simulink library "AEMS_Standard_Library"  (R2016b)
settings: Solver=ode45  StartTime=0.0  StopTime=10.0  RelTol=1e-3
undefined symbols (not defined in the file or in its folder): BkPY, carto, Cbx_extegr, Cbx_lpegrsys, Cbx_portegr, Cnx_bnk_nr_conf, Cnx_cyl_nr_conf, ConfigManagement, configuration_management, Cxx_dcm_io_tmr_end_xxxx, Cxx_dcm_rt_tmr_end, Cxx_DID_xxxx_IO_max, Cxx_DID_xxxx_IO_min, Cxx_egrhsofs, Cxx_vmaniegi, DEM_DEBOUNCE_FREEZE, DEM_DTR_CTL_INVISIBLE, DEM_DTR_CTL_NORMAL, Dem_DtrId2_XXX, Dem_DtrId3_XXX, Dem_DtrId4_XXX, Dem_DtrId5_XXX, Dem_DtrId6_XXX, Dem_DtrId7_XXX, Dem_DtrId8_XXX, Dem_DtrId9_XXX, Dem_DtrId_XXX, Dem_EnableConditionId2_XXX, Dem_EnableConditionId3_XXX, Dem_EnableConditionId4_XXX, Dem_EnableConditionId5_XXX, Dem_EnableConditionId6_XXX, Dem_EnableConditionId7_XXX, Dem_EnableConditionId8_XXX, Dem_EnableConditionId_XXX, Dem_EventId, Dem_EventId2_XXX, Dem_EventId3_XXX, Dem_EventId4_XXX, Dem_EventId5_XXX, Dem_EventId6_XXX, Dem_EventId7_XXX, Dem_EventId8_XXX, Dem_EventId9_XXX, Dem_EventId_Device_Faulttype, Dem_EventId_XXX, DEM_IUMPR_GENERAL_DENOMINATOR, DEM_OPCYC_IGNITION, Dem_RatioId2_XXX, Dem_RatioId3_XXX, Dem_RatioId4_XXX, Dem_RatioId5_XXX, Dem_RatioId6_XXX, Dem_RatioId7_XXX, Dem_RatioId8_XXX, Dem_RatioId_XXX, Dem_StorageConditionId2_XXX, Dem_StorageConditionId3_XXX, Dem_StorageConditionId4_XXX, Dem_StorageConditionId5_XXX ... (+65)
libraries: AEMS_Standard_Library x477, simulink x2
(part 6 of 39)

== system AEMS_Standard_Library/DEM ==
  note: AUTOSAR IN
  note: AUTOSAR OUT
  note: FIM
  note: NISSAN USES
  AEMS_DEM_COUNTER_BASED_DEBOUNCE : Subsystem  Tag=[LIB]  Description=This subsystem is interface for self diagnosis standard calculated from similar condition and NG judgment.  mask(AEMS_DEM_COUNTER_BASED_DEBOUNCE){eventid=Dem_EventId_Device_Faulttype, Specificchoix=off, Dim_num=1, DemDebounceBehavior1=DEM_DEBOUNCE_FREEZE (0), DemDebounceBehavior2=DEM_DEBOUNCE_FREEZE (0), DemDebounceBehavior3=DEM_DEBOUNCE_FREEZE (0), DemDebounceBehavior4=DEM_DEBOUNCE_FREEZE (0), DemDebounceBehavior5=DEM_DEBOUNCE_FREEZE (0), DemDebounceBehavior6=DEM_DEBOUNCE_FREEZE (0), DemDebounceBehavior7=DEM_DEBOUNCE_FREEZE (0), DemDebounceBehavior8=DEM_DEBOUNCE_FREEZE (0), DemCounterFailedThreshold=Cnx_dem_fail_thd_Device_Faulttype, DemCounterIncrementStepSize=Cnx_dem_pfail_inc_step_Device_Faulttype, DemCounterJumpUp=Cbx_dem_jmp_up_act_Device_Faulttype, DemCounterJumpUpValue=Cnx_dem_jmp_up_pfail_Device_Faulttype, DemCounterPassedThreshold=Cnx_dem_pass_thd_Device_Faulttype, DemCounterDecrementStepSize=Cnx_dem_ppass_dec_step_Device_Faulttype, DemCounterJumpDown=Cbx_dem_jmp_dwn_act_Device_Faulttype, DemCounterJumpDownValue=Cnx_dem_jmp_dwn_ppass_Device_Faulttype, DemCounterBypassFailure=Cbx_dem_byp_fail_Device_Faulttype, ToDataStoreMemory=off}
      mask prompts: eventid "Identifier of a diagnostic event (EventId)"; Specificchoix "Specific case used only for Nissan cases"; Dim_num "Dimension :"; DemDebounceBehavior1 "Dem Debounce Behavior 1"; DemDebounceBehavior2 "Dem Debounce Behavior 2"; DemDebounceBehavior3 "Dem Debounce Behavior 3"; DemDebounceBehavior4 "Dem Debounce Behavior 4"; DemDebounceBehavior5 "Dem Debounce Behavior 5"; DemDebounceBehavior6 "Dem Debounce Behavior 6"; DemDebounceBehavior7 "Dem Debounce Behavior 7"; DemDebounceBehavior8 "Dem Debounce Behavior 8"; DemCounterFailedThreshold "Dem Debounce Counter Failed Threshold"; DemCounterIncrementStepSize "Dem Debounce Counter Increment Step Size"; DemCounterJumpUp "Dem Debounce Counter Jump Up"; DemCounterJumpUpValue "Dem Debounce Counter Jump Up Value"; DemCounterPassedThreshold "Dem Debounce Counter Passed Threshold"; DemCounterDecrementStepSize "Dem Debounce Counter Decrement Step Size"; DemCounterJumpDown "Dem Debounce Counter Jump Down"; DemCounterJumpDownValue "Dem Debounce Counter Jump Down Value"; DemCounterBypassFailure "Dem Debounce Counter Bypass Failure"; ToDataStoreMemory "Write Output To Data Store Memory"
      mask help:
      | It  transmit the status Failed or Passed to the DEM. Accordingly, some bits of the UDS DTC status byte changes synchronously or asynchronously according to the configuration. Debounce is based on counter.
      |
      | -INPUTS-
      | conditionfulfilled: specifies whether the storage condition assigned to the StorageConditionId is fulfilled
      | prefailed: Monitor reports nonqualified test result pre-failed
      | prepassed: Monitor reports nonqualified test result pre-passed
      | ClearDataRequest:Clears the Data Request value
      | reseteventdebounce: Freeze or reset the internal debounce counter/timer.
      |
      | -OUTPUTS-
      | debouncevalue: Value of the debounce counter
      | failed: Diagnostic monitor reports an event Failed
      | passed: Diagnostic monitor reports an event passed
      |
      | -PARAMETERS-
      | Device: Device type
      | FaultType: Fault Type
      | EventId: Internal identifier of a diagnostic event. 0 is not a valid value.
      | Dem Debounce Behavior: The event debounce counter will be frozen or reset (0 for FREEZE and 1 for RESET)
      | Dem Debounce Counter Failed Threshold: Defines the value of the internal debounce counter, which indicates the failed status.
      | Dem Debounce Counter Increment Step Size: Defines the incrementation  step size for counter (PREFAILED)
      | Dem Debounce Counter Jump Up: Activation of Jump-Up. True: activated. False: deactivated
      | Dem Debounce Counter Jump Up Value: Initialization value for the counter when PREFAILED
      | Dem Debounce Counter Passed Threshold: Defines the value of the internal debounce counter, which indicates the passed status.
      | Dem Debounce Counter Decrement Step Size: Defines the decrementation step for of counter (PREPASSED).
      | Dem Debounce Counter Jump Down: Activation of Jump-Down. True: Jump-Down activated
      | Dem Debounce Counter Jump Down Value: Initialization value for the counter when PREPASSED
      mask init:
      | lib_path = gcb;
      | child_lib = find_system(lib_path,'LookUnderMasks','all','FollowLinks','on','Name','AEMS_DEM_COUNTER_BASED_DEBOUNCE_D');
      | Attribute_Format_String_Part1 = '%<MaskType>\n EventId : = %<eventid> \n Specific case used only for Nissan cases := %<Specificchoix> ';
      | Attribute_Format_String_Part2 = '';
      | if strcmpi(Specificchoix,'off')
      |     Dim_num = '1';
      | else
      |     Attribute_Format_String_Part2 = '\n Dimension := %<Dim_num> ';
      | end
      | dim_block = ['AEMS_DEM_COUNTER_BASED_DEBOUNCE_' Dim_num 'D'];
      | 
      | rep_block = ['AEMS_Standard_Library/SUB/',dim_block];
      | if ismember(get_param(child_lib,'MaskType'),{dim_block})
      | else
      |     replace_block(lib_path,'FollowLinks','on','Name','AEMS_DEM_COUNTER_BASED_DEBOUNCE_D',rep_block,'noprompt');
      | end
      | 
      | Attribute_Format_String_Part3='';
      | for i=1:str2num(Dim_num)
      |     Attribute_Format_String_Part3=[Attribute_Format_String_Part3,'\n Dem Debounce Behavior ',num2str(i),' := %<DemDebounceBehavior',num2str(i),'>'];
      |     set_param([child_lib{:}],['DemDebounceBehavior',num2str(i)],get_param(lib_path,['DemDebounceBehavior',num2str(i)]));
      | end
      | 
      | if 1
      |     DemCounterFailedThreshold_tmp = get_param(lib_path,'DemCounterFailedThreshold');
      |     DemCounterIncrementStepSize_tmp = get_param(lib_path,'DemCounterIncrementStepSize');
      |     DemCounterJumpUp_tmp = get_param(lib_path,'DemCounterJumpUp');
      |     DemCounterJumpUpValue_tmp = get_param(lib_path,'DemCounterJumpUpValue');
      |     DemCounterPassedThreshold_tmp = get_param(lib_path,'DemCounterPassedThreshold');
      |     DemCounterDecrementStepSize_tmp = get_param(lib_path,'DemCounterDecrementStepSize');
      |     DemCounterJumpDown_tmp = get_param(lib_path,'DemCounterJumpDown');
      |     DemCounterJumpDownValue_tmp = get_param(lib_path,'DemCounterJumpDownValue');
      |     DemCounterBypassFailure_tmp = get_param(lib_path,'DemCounterBypassFailure');
      |     
      |     set_param([child_lib{:}],'eventid',eventid);
      |     set_param([child_lib{:}],'DemCounterFailedThreshold',DemCounterFailedThreshold_tmp);
      |     set_param([child_lib{:}],'DemCounterIncrementStepSize',DemCounterIncrementStepSize_tmp);
      |     set_param([child_lib{:}],'DemCounterJumpUp',DemCounterJumpUp_tmp);
      |     set_param([child_lib{:}],'DemCounterJumpUpValue',DemCounterJumpUpValue_tmp);
      |     set_param([child_lib{:}],'DemCounterPassedThreshold',DemCounterPassedThreshold_tmp);
      |     set_param([child_lib{:}],'DemCounterDecrementStepSize',DemCounterDecrementStepSize_tmp);
      |     set_param([child_lib{:}],'DemCounterJumpDown',DemCounterJumpDown_tmp);
      |     set_param([child_lib{:}],'DemCounterJumpDownValue',DemCounterJumpDownValue_tmp);
      |     set_param([child_lib{:}],'DemCounterBypassFailure',DemCounterBypassFailure_tmp);
      | else
      |     %do nothing
      | end
      | 
      | %If To DataStoreMemory is enabled...
      | 
      | if strcmpi(ToDataStoreMemory,'on')&& isempty(find_system(lib_path,'LookUnderMasks','all','FollowLinks','on','Name','AEMS_SRFLIPFLOP'))
      |     add_block('AEMS_Standard_Library/FLAG/AEMS_SRFLIPFLOP',[lib_path,'/AEMS_SRFLIPFLOP'],'Position',[995 224 1080 346]);
      |     add_block('simulink/Signal Attributes/Data Type Conversion',[lib_path,'/Data Type Conversion'],'Position',[1145 273 1200 297],'ShowName','off');
      |     add_block('simulink/Signal Routing/Data Store Write',[lib_path,'/Data Store Write'],'Position',[1250 272 1475 298],'ShowName','off');
      |     add_line(lib_path,'AEMS_DEM_COUNTER_BASED_DEBOUNCE_D/2','AEMS_SRFLIPFLOP/1','AutoRouting','on');
      |     add_line(lib_path,'AEMS_DEM_COUNTER_BASED_DEBOUNCE_D/3','AEMS_SRFLIPFLOP/2','AutoRouting','on');
      |     add_line(lib_path,'AEMS_SRFLIPFLOP/1','Data Type Conversion/1');
      |     add_line(lib_path,'Data Type Conversion/1','Data Store Write/1');
      | elseif strcmpi(ToDataStoreMemory,'off') && ~isempty(find_system(lib_path,'LookUnderMasks','all','FollowLinks','on','Name','AEMS_SRFLIPFLOP'))
      |     delete_block([lib_path,'/Data Type Conversion']);
      |     delete_block([lib_path,'/Data Store Write']);
      |     delete_block([lib_path,'/AEMS_SRFLIPFLOP']);
      |     delete_line(find_system(lib_path,'FollowLinks','on','FindAll','on','LookUnderMasks','on','Type','line','Connected','off'));
      | end
      | if strcmpi(ToDataStoreMemory,'on')
      |     %Get Task Rate of this block.(As per AEMS arch, all the blks shall be
      |     %kept under the runnable. The Runnable name will ncontain the sample
      |     %time suffix. From where we can get it.
      |     model_type_pos = strsplit(lib_path,'/');%to split all the layer paths in order to get the runnable path
      |     runnable_path = [bdroot '/' model_type_pos{2}];%to get the runnable or AIPCALL path
      |     trg_port_name = get_param(find_system(runnable_path,'BlockType','TriggerPort'),'Name');%to get the function call trigger name
      |     TaskRate = '';%the raster suffix is stored in the parameter
      |     
      |     if ~isempty(trg_port_name)
      |         trg_port_name_spltd = strsplit(trg_port_name{1},'_');%splitting is done in order to get the raster and its type(Sched or Event)
      |         
      |         % checking for rasters of type Sched or Event especially occuring in
      |         % runnables
      |         if ~isempty(regexp(trg_port_name_spltd{1},'^Sched|^Event','once'))
      |             TaskRate = ['_' regexprep(trg_port_name_spltd{1},'Sched|Event','','once')];
      |             
      |             %checking if the raster is dcmcb and this is applicable only for
      |             %APICALL
      |         elseif ~isempty(regexp([trg_port_name_spltd{1} '_' trg_port_name_spltd{2} '_' ],'^DataServices_DCM_|^RoutineServices_DCM_','once'))||...
      |                 ~isempty(regexp(trg_port_name_spltd{1},'^Dcm$','once'))
      |             TaskRate = '_dcmcb';
      |             
      |             %checking if this block is used under the function call trigger
      |             %starting with "Com" and then giving an error message
      |             %this is applicable only for APICALL
      |         elseif ~isempty(regexp(trg_port_name_spltd{1},'^Com$','once'))
      |             msg = sprintf(['\n','The FIM block "' lib_path '" should not be present within APICALLs having function call trigger as "Com"']);
      |             errordlg(msg);
      |             return;
      |         end
      |     end
      |     DataStoreName = [eventid,TaskRate];
      |     set_param([lib_path,'/Data Store Write'],'DataStoreName',DataStoreName);
      | end
      | 
      | Attribute_Format_String_Part5 = '\n Write Output To Data Store Memory := %<ToDataStoreMemory>';
      | 
      | Attribute_Format_String_Part4='\n Dem Debounce Counter Failed Threshold := %<DemCounterFailedThreshold>\nDem Debounce Counter Increment Step Size := %<DemCounterIncrementStepSize>\nDem Debounce Counter Jump Up := %<DemCounterJumpUp>\nDem Debounce Counter Jump Up Value := %<DemCounterJumpUpValue>\nDem Debounce Counter Passed Threshold := %<DemCounterPassedThreshold>\nDem Debounce Counter Decrement Step Size := %<DemCounterDecrementStepSize>\nDem Debounce Counter Jump Down := %<DemCounterJumpDown>\nDem Debounce Counter Jump Down Value := %<DemCounterJumpDownValue>\nDem Debounce Counter Bypass Failure = %<DemCounterBypassFailure>';
      | Attribute_Format_String = [Attribute_Format_String_Part1,Attribute_Format_String_Part2,Attribute_Format_String_Part3,Attribute_Format_String_Part4, Attribute_Format_String_Part5];
      | set_param(lib_path,'AttributesFormatString',Attribute_Format_String);
      settings: AttributesFormatString=%<MaskType>\n EventId : = %<eventid> \n Specific case used only for Nissan cases := %<Specificchoix> \n Dem Debounce Behavior 1 := %<DemDebounceBehavior1>\n Dem Debounce Counter Failed Threshold := %<DemCounterFailedThreshold>\nDem Debounce Counter Increment Step Size := %<DemCounterIncrementStepSize>\nDem Debounce Counter Jump Up := %<DemCounterJumpUp>\nDem Debounce Counter Jump Up Value := %<DemCounterJumpUpValue>\nDem Debounce Counter Passed Threshold := %<DemCounterPassedThreshold>\nDem Debounce Counter Decrement Step Size := %<DemCounterDecrementStepSize>\nDem Debounce Counter Jump Down := %<DemCounterJumpDown>\nDem Debounce Counter Jump Down Value := %<DemCounterJumpDownValue>\nDem Debounce Counter Bypass Failure = %<DemCounterBypassFailure>\n Write Output To Data Store Memory := %<ToDataStoreMemory>
      mask Help:
      | eval('path_lib=fileparts(which(''AEMS_Standard_Library''));');
      | doc_path = [path_lib '\help\AEMS_DEM_COUNTER_BASED_DEBOUNCE.pdf'];
      | eval('open(doc_path)');
      mask Callback eventid:
      | lib_path=gcb;
      | EventID=get_param(lib_path,'eventid');
      | Splitname=regexp(EventID,'_','all');
      | EventID_Name=extractAfter(EventID,EventID(1:Splitname(2)));
      | 
      | Fail_Thrs=strcat('Cnx_dem_fail_thd_',EventID_Name);
      | set_param(lib_path,'DemCounterFailedThreshold',Fail_Thrs);
      | 
      | Inc_size=strcat('Cnx_dem_pfail_inc_step_',EventID_Name);
      | set_param(lib_path,'DemCounterIncrementStepSize',Inc_size);
      | 
      | Jumpup=strcat('Cbx_dem_jmp_up_act_',EventID_Name);
      | set_param(lib_path,'DemCounterJumpUp',Jumpup);
      | 
      | Jumpup_value=strcat('Cnx_dem_jmp_up_pfail_',EventID_Name);
      | set_param(lib_path,'DemCounterJumpUpValue',Jumpup_value);
      | 
      | Pass_Thrs=strcat('Cnx_dem_pass_thd_',EventID_Name);
      | set_param(lib_path,'DemCounterPassedThreshold',Pass_Thrs);
      | 
      | Dec_size=strcat('Cnx_dem_ppass_dec_step_',EventID_Name);
      | set_param(lib_path,'DemCounterDecrementStepSize',Dec_size);
      | 
      | Jumpdown=strcat('Cbx_dem_jmp_dwn_act_',EventID_Name);
      | set_param(lib_path,'DemCounterJumpDown',Jumpdown);
      | 
      | Jumpdown_value=strcat('Cnx_dem_jmp_dwn_ppass_',EventID_Name);
      | set_param(lib_path,'DemCounterJumpDownValue',Jumpdown_value);
      | 
      | BypassFailure=strcat('Cbx_dem_byp_fail_',EventID_Name);
      | set_param(lib_path,'DemCounterBypassFailure',BypassFailure);
      | 
      | ToDataStoreMemory = get_param(lib_path,'ToDataStoreMemory');
      | 
      | if strcmpi(ToDataStoreMemory,'on')
      | model_type_pos = strsplit(lib_path,'/');%to split all the layer paths in order to get the runnable path
      | runnable_path = [bdroot '/' model_type_pos{2}];%to get the runnable or AIPCALL path
      | trg_port_name = get_param(find_system(runnable_path,'BlockType','TriggerPort'),'Name');%to get the function call trigger name
      | TaskRate = '';%the raster suffix is stored in the parameter
      | 
      | if ~isempty(trg_port_name)
      |     trg_port_name_spltd = strsplit(trg_port_name{1},'_');%splitting is done in order to get the raster and its type(Sched or Event)
      | 
      |     % checking for rasters of type Sched or Event especially occuring in
      |     % runnables
      |     if ~isempty(regexp(trg_port_name_spltd{1},'^Sched\d+(ms|s)$|^Event+(sync|knock|comc|coml|dcmcb)$','once'))
      |         TaskRate = ['_' regexp(trg_port_name_spltd{1},'\d+(ms|s)$|sync$|knock$|comc$|coml$|dcmcb$','match','once')];
      | 
      |     %checking if the raster is dcmcb and this is applicable only for
      |     %APICALL
      |     elseif ~isempty(regexp([trg_port_name_spltd{1} '_' trg_port_name_spltd{2} '_' ],'^DataServices_DCM_|^RoutineServices_DCM_','once'))||...
      |             ~isempty(regexp(trg_port_name_spltd{1},'^Dcm$','once'))
      |         TaskRate = '_dcmcb';
      | 
      |     %checking if this block is used under the function call trigger
      |     %starting with "Com" and then giving an error message
      |     %this is applicable only for APICALL
      |     elseif ~isempty(regexp(trg_port_name_spltd{1},'^Com$','once'))
      |         msg = sprintf(['\n','The DEM blocks "' Thisblk '" should not be present within APICALLs having function call trigger as "Com"']);
      |         errordlg(msg);
      |         return;
      |     end
      | end
      | DataStoreName = [EventID TaskRate];%the variable name that should be given to DataStoreRead block
      | set_param([lib_path,'/Data Store Write'],'DataStoreName',DataStoreName);
      | else
      |     %do nothing
      | end
      mask Callback Specificchoix:
      | Outputs_From_get_param = get_param(gcb,'Dim_num');
      | Specificchoice_get_param = get_param(gcb,'Specificchoix');
      | maskobj = Simulink.Mask.get(gcbh);
      | maskobj_param = maskobj.Parameters;
      |     if strcmpi(Specificchoice_get_param,'on')
      |        Non=4;
      |         maskobj_param(3).Visible = 'on';
      |         maskobj_param(3).Enabled = 'on';
      |         switch(Outputs_From_get_param)
      |             case '1'
      |                 Non=4;
      |             case '2'
      |                 Non=5;
      |             case '3'
      |                 Non=6;
      |              case '4'
      |                  Non=7;
      |              case '6'
      |                  Non=9;
      |              case '8'
      |                  Non=11;
      |         end
      |     else
      |         maskobj_param(3).Visible = 'off';
      |         maskobj_param(3).Enabled = 'off';
      |         Non=4;
      |     end
      | for i=4:Non
      |     maskobj_param(i).Visible = 'on';
      |     maskobj_param(i).Enabled = 'on';
      | end
      | for i=Non+1:11
      |     maskobj_param(i).Visible = 'off';
      |     maskobj_param(i).Enabled = 'off';
      | end
      | clear maskobj_param;
      | clear maskobj;
      mask TypeOptions Dim_num: 1 | 2 | 3 | 4 | 6 | 8
      mask Callback Dim_num:
      | Outputs_From_get_param = get_param(gcb,'Dim_num');
      | Specificchoice_get_param = get_param(gcb,'Specificchoix');
      | maskobj = Simulink.Mask.get(gcbh);
      | maskobj_param = maskobj.Parameters;
      |     if strcmpi(Specificchoice_get_param,'on')
      |        Non=4;
      |         maskobj_param(3).Visible = 'on';
      |         maskobj_param(3).Enabled = 'on';
      |         switch(Outputs_From_get_param)
      |             case '1'
      |                 Non=4;
      |             case '2'
      |                 Non=5;
      |             case '3'
      |                 Non=6;
      |              case '4'
      |                  Non=7;
      |              case '6'
      |                  Non=9;
      |              case '8'
      |                  Non=11;
      |         end
      |     else
      |         maskobj_param(3).Visible = 'off';
      |         maskobj_param(3).Enabled = 'off';
      |         Non=4;
      |     end
      | for i=4:Non
      |     maskobj_param(i).Visible = 'on';
      |     maskobj_param(i).Enabled = 'on';
      | end
      | for i=Non+1:11
      |     maskobj_param(i).Visible = 'off';
      |     maskobj_param(i).Enabled = 'off';
      | end
      | clear maskobj_param;
      | clear maskobj;
      mask TypeOptions DemDebounceBehavior1: DEM_DEBOUNCE_FREEZE (0) | DEM_DEBOUNCE_RESET (1)
      mask TypeOptions DemDebounceBehavior2: DEM_DEBOUNCE_FREEZE (0) | DEM_DEBOUNCE_RESET (1)
      mask TypeOptions DemDebounceBehavior3: DEM_DEBOUNCE_FREEZE (0) | DEM_DEBOUNCE_RESET (1)
      mask TypeOptions DemDebounceBehavior4: DEM_DEBOUNCE_FREEZE (0) | DEM_DEBOUNCE_RESET (1)
      mask TypeOptions DemDebounceBehavior5: DEM_DEBOUNCE_FREEZE (0) | DEM_DEBOUNCE_RESET (1)
      mask TypeOptions DemDebounceBehavior6: DEM_DEBOUNCE_FREEZE (0) | DEM_DEBOUNCE_RESET (1)
      mask TypeOptions DemDebounceBehavior7: DEM_DEBOUNCE_FREEZE (0) | DEM_DEBOUNCE_RESET (1)
      mask TypeOptions DemDebounceBehavior8: DEM_DEBOUNCE_FREEZE (0) | DEM_DEBOUNCE_RESET (1)
  AEMS_DEM_COUNTER_BASED_DEBOUNCE_THRSHOLD_DYN : Subsystem  Tag=[LIB]  Description=This subsystem is interface for self diagnosis standard calculated from similar condition and NG judgment.  mask(AEMS_DEM_COUNTER_BASED_DEBOUNCE_THRSHOLD_DYN){eventid=Dem_EventId_Device_Faulttype, Specificchoix=off, Dim_num=1, DemDebounceBehavior1=DEM_DEBOUNCE_FREEZE (0), DemDebounceBehavior2=DEM_DEBOUNCE_RESET (1), DemDebounceBehavior3=DEM_DEBOUNCE_FREEZE (0), DemDebounceBehavior4=DEM_DEBOUNCE_FREEZE (0), DemDebounceBehavior5=DEM_DEBOUNCE_RESET (1), DemDebounceBehavior6=DEM_DEBOUNCE_FREEZE (0), DemDebounceBehavior7=DEM_DEBOUNCE_RESET (1), DemDebounceBehavior8=DEM_DEBOUNCE_FREEZE (0), DemCounterIncrementStepSize=Cnx_dem_pfail_inc_step_Device_Faulttype, DemCounterJumpUp=Cbx_dem_jmp_up_act_Device_Faulttype, DemCounterJumpUpValue=Cnx_dem_jmp_up_pfail_Device_Faulttype, DemCounterDecrementStepSize=Cnx_dem_ppass_dec_step_Device_Faulttype, DemCounterJumpDown=Cbx_dem_jmp_dwn_act_Device_Faulttype, DemCounterJumpDownValue=Cnx_dem_jmp_dwn_ppass_Device_Faulttype, DemCounterBypassFailure=Cbx_dem_byp_fail_Device_Faulttype, ToDataStoreMemory=on}
      mask prompts: eventid "Identifier of a diagnostic event (EventId)"; Specificchoix "Specific case used only for Nissan cases"; Dim_num "Counter_Based_Debounce_Thrshold_Dyn_Dimention"; DemDebounceBehavior1 "Dem Debounce Behavior 1"; DemDebounceBehavior2 "Dem Debounce Behavior 2"; DemDebounceBehavior3 "Dem Debounce Behavior 3"; DemDebounceBehavior4 "Dem Debounce Behavior 4"; DemDebounceBehavior5 "Dem Debounce Behavior 5"; DemDebounceBehavior6 "Dem Debounce Behavior 6"; DemDebounceBehavior7 "Dem Debounce Behavior 7"; DemDebounceBehavior8 "Dem Debounce Behavior 8"; DemCounterIncrementStepSize "Dem Debounce Counter Increment Step Size"; DemCounterJumpUp "Dem Debounce Counter Jump Up"; DemCounterJumpUpValue "Dem Debounce Counter Jump Up Value"; DemCounterDecrementStepSize "Dem Debounce Counter Decrement Step Size"; DemCounterJumpDown "Dem Debounce Counter Jump Down"; DemCounterJumpDownValue "Dem Debounce Counter Jump Down Value"; DemCounterBypassFailure "Dem Debounce Counter Bypass Failure"; ToDataStoreMemory "Write Output To Data Store Memory"
      mask help:
      | It  transmit the status Failed or Passed to the DEM. Accordingly, some bits of the UDS DTC status byte changes synchronously or asynchronously according to the configuration. Debounce is based on counter.
      |
      | -INPUTS-
      | conditionfulfilled: specifies whether the storage condition assigned to the StorageConditionId is fulfilled
      | prefailed: Monitor reports nonqualified test result pre-failed
      | prepassed: Monitor reports nonqualified test result pre-passed
      | failedthreshold: Defines the value of the internal debounce counter, which indicates the failed status.
      | passedthreshold: Defines the value of the internal debounce counter, which indicates the passed status.
      | ClearDataRequest:Clears the Data Request value
      | reseteventdebounce: Freeze or reset the internal debounce counter/timer.
      |
      | -OUTPUTS-
      | debouncevalue: Value of the debounce counter
      | failed: Diagnostic monitor reports an event Failed
      | passed: Diagnostic monitor reports an event passed
      |
      | -PARAMETERS-
      | EventId: Internal identifier of a diagnostic event. 0 is not a valid value.
      | Dem Debounce Behavior: The event debounce counter will be frozen or reset (0 for FREEZE and 1 for RESET)
      | Dem Debounce Counter Increment Step Size: Defines the incrementation  step size for counter (PREFAILED)
      | Dem Debounce Counter Jump Up: Activation of Jump-Up. True: activated. False: deactivated
      | Dem Debounce Counter Jump Up Value: Initialization value for the counter when PREFAILED
      | Dem Debounce Counter Decrement Step Size: Defines the decrementation step for of counter (PREPASSED).
      | Dem Debounce Counter Jump Down: Activation of Jump-Down. True: Jump-Down activated
      | Dem Debounce Counter Jump Down Value: Initialization value for the counter when PREPASSED
      mask init:
      | lib_path = gcb;
      | child_lib = find_system(lib_path,'LookUnderMasks','all','FollowLinks','on','Name','AEMS_DEM_COUNTER_BASED_DEBOUNCE_THRSHOLD_DYN_D');
      | Attribute_Format_String_Part1 = '%<MaskType>\n EventId : %<eventid> \n Specific case used only for Nissan cases = %<Specificchoix> ';
      | Attribute_Format_String_Part2 = '';
      | if strcmpi(Specificchoix,'off')
      |    Dim_num = '1';
      | else
      |    Attribute_Format_String_Part2 = '\n Counter_Based_Debounce_Thrshold_Dyn_Dimention = %<Dim_num> '; 
      | end
      | dim_block = ['AEMS_DEM_COUNTER_BASED_DEBOUNCE_THRSHOLD_DYN_' Dim_num 'D'];
      | 
      | rep_block = ['AEMS_Standard_Library/SUB/',dim_block];
      | if ismember(get_param(child_lib,'MaskType'),{dim_block})
      | else
      |     replace_block(lib_path,'FollowLinks','on','Name','AEMS_DEM_COUNTER_BASED_DEBOUNCE_THRSHOLD_DYN_D',rep_block,'noprompt');
      | end
      | 
      | Attribute_Format_String_Part3='';
      | for i=1:str2num(Dim_num)
      |     Attribute_Format_String_Part3=[Attribute_Format_String_Part3,'\n Dem Debounce Behavior ',num2str(i),' = %<DemDebounceBehavior',num2str(i),'>'];
      |     set_param([child_lib{:}],['DemDebounceBehavior',num2str(i)],get_param(lib_path,['DemDebounceBehavior',num2str(i)]));
      | end
      |     
      | DemCounterIncrementStepSize_tmp = get_param(lib_path,'DemCounterIncrementStepSize');
      | DemCounterJumpUp_tmp = get_param(lib_path,'DemCounterJumpUp');
      | DemCounterJumpUpValue_tmp = get_param(lib_path,'DemCounterJumpUpValue');
      | DemCounterDecrementStepSize_tmp = get_param(lib_path,'DemCounterDecrementStepSize');
      | DemCounterJumpDown_tmp = get_param(lib_path,'DemCounterJumpDown');
      | DemCounterJumpDownValue_tmp = get_param(lib_path,'DemCounterJumpDownValue');
      | DemCounterBypassFailure_tmp = get_param(lib_path,'DemCounterBypassFailure');
      | 
      | set_param([child_lib{:}],'eventid',eventid);
      | set_param([child_lib{:}],'DemCounterIncrementStepSize',DemCounterIncrementStepSize_tmp);
      | set_param([child_lib{:}],'DemCounterJumpUp',DemCounterJumpUp_tmp);
      | set_param([child_lib{:}],'DemCounterJumpUpValue',DemCounterJumpUpValue_tmp);
      | set_param([child_lib{:}],'DemCounterDecrementStepSize',DemCounterDecrementStepSize_tmp);
      | set_param([child_lib{:}],'DemCounterJumpDown',DemCounterJumpDown_tmp);
      | set_param([child_lib{:}],'DemCounterJumpDownValue',DemCounterJumpDownValue_tmp);
      | set_param([child_lib{:}],'DemCounterBypassFailure',DemCounterBypassFailure_tmp);
      | 
      | %If To DataStoreMemory is enabled...
      | if strcmpi(ToDataStoreMemory,'on') && isempty(find_system(lib_path,'LookUnderMasks','all','FollowLinks','on','Name','AEMS_SRFLIPFLOP'))
      |    add_block('AEMS_Standard_Library/FLAG/AEMS_SRFLIPFLOP',[lib_path,'/AEMS_SRFLIPFLOP'],'Position',[1020 209 1105 331]);
      |    add_block('simulink/Signal Attributes/Data Type Conversion',[lib_path,'/Data Type Conversion'],'Position',[1140 258 1195 282],'ShowName','off')
      |    add_block('simulink/Signal Routing/Data Store Write',[lib_path,'/Data Store Write'],'Position',[1250 257 1475 283],'ShowName','off');
      |    add_line(lib_path,'AEMS_DEM_COUNTER_BASED_DEBOUNCE_THRSHOLD_DYN_D/2','AEMS_SRFLIPFLOP/1','AutoRouting','on');
      |    add_line(lib_path,'AEMS_DEM_COUNTER_BASED_DEBOUNCE_THRSHOLD_DYN_D/3','AEMS_SRFLIPFLOP/2','AutoRouting','on');
      |    add_line(lib_path,'AEMS_SRFLIPFLOP/1','Data Type Conversion/1');
      |    add_line(lib_path,'Data Type Conversion/1','Data Store Write/1');
      | elseif strcmpi(ToDataStoreMemory,'off') && ~isempty(find_system(lib_path,'LookUnderMasks','all','FollowLinks','on','Name','AEMS_SRFLIPFLOP'))
      |    delete_block([lib_path,'/AEMS_SRFLIPFLOP']);
      |    delete_block([lib_path,'/Data Type Conversion']);
      |    delete_block([lib_path,'/Data Store Write']);
      |    delete_line(find_system(lib_path,'FollowLinks','on','FindAll','on','LookUnderMasks','on','Type','line','Connected','off'));
      | end
      | 
      | if strcmpi(ToDataStoreMemory,'on')
      |     %Get Task Rate of this block.(As per AEMS arch, all the blks shall be
      |     %kept under the runnable. The Runnable name will ncontain the sample
      |     %time suffix. From where we can get it.
      |     model_type_pos = strsplit(lib_path,'/');%to split all the layer paths in order to get the runnable path
      |     runnable_path = [bdroot '/' model_type_pos{2}];%to get the runnable or AIPCALL path
      |     trg_port_name = get_param(find_system(runnable_path,'BlockType','TriggerPort'),'Name');%to get the function call trigger name
      |     TaskRate = '';%the raster suffix is stored in the parameter
      |     
      |     if ~isempty(trg_port_name)
      |         trg_port_name_spltd = strsplit(trg_port_name{1},'_');%splitting is done in order to get the raster and its type(Sched or Event)
      |         
      |         % checking for rasters of type Sched or Event especially occuring in
      |         % runnables
      |         if ~isempty(regexp(trg_port_name_spltd{1},'^Sched|^Event','once'))
      |             TaskRate = ['_' regexprep(trg_port_name_spltd{1},'Sched|Event','','once')];
      |             
      |             %checking if the raster is dcmcb and this is applicable only for
      |             %APICALL
      |         elseif ~isempty(regexp([trg_port_name_spltd{1} '_' trg_port_name_spltd{2} '_' ],'^DataServices_DCM_|^RoutineServices_DCM_','once'))||...
      |                 ~isempty(regexp(trg_port_name_spltd{1},'^Dcm$','once'))
      |             TaskRate = '_dcmcb';
      |             
      |             %checking if this block is used under the function call trigger
      |             %starting with "Com" and then giving an error message
      |             %this is applicable only for APICALL
      |         elseif ~isempty(regexp(trg_port_name_spltd{1},'^Com$','once'))
      |             msg = sprintf(['\n','The FIM block "' lib_path '" should not be present within APICALLs having function call trigger as "Com"']);
      |             errordlg(msg);
      |             return;
      |         end
      |     end
      |     DataStoreName = [eventid,TaskRate];
      |     set_param([lib_path,'/Data Store Write'],'DataStoreName',DataStoreName);
      | end
      | 
      | Attribute_Format_String_Part5 = '\n Write Output To Data Store Memory := %<ToDataStoreMemory>';
      | 
      | Attribute_Format_String_Part4='\n Dem Debounce Counter Increment Step Size = %<DemCounterIncrementStepSize>\nDem Debounce Counter Jump Up = %<DemCounterJumpUp>\nDem Debounce Counter Jump Up Value = %<DemCounterJumpUpValue>\nDem Debounce Counter Decrement Step Size = %<DemCounterDecrementStepSize>\nDem Debounce Counter Jump Down = %<DemCounterJumpDown>\nDem Debounce Counter Jump Down Value = %<DemCounterJumpDownValue>\nDem Debounce Counter Bypass Failure = %<DemCounterBypassFailure>';
      | Attribute_Format_String = [Attribute_Format_String_Part1,Attribute_Format_String_Part2,Attribute_Format_String_Part3,Attribute_Format_String_Part4, Attribute_Format_String_Part5];
      | set_param(lib_path,'AttributesFormatString',Attribute_Format_String);
      settings: AttributesFormatString=%<MaskType>\n EventId : %<eventid> \n Specific case used only for Nissan cases = %<Specificchoix> \n Dem Debounce Behavior 1 = %<DemDebounceBehavior1>\n Dem Debounce Counter Increment Step Size = %<DemCounterIncrementStepSize>\nDem Debounce Counter Jump Up = %<DemCounterJumpUp>\nDem Debounce Counter Jump Up Value = %<DemCounterJumpUpValue>\nDem Debounce Counter Decrement Step Size = %<DemCounterDecrementStepSize>\nDem Debounce Counter Jump Down = %<DemCounterJumpDown>\nDem Debounce Counter Jump Down Value = %<DemCounterJumpDownValue>\nDem Debounce Counter Bypass Failure = %<DemCounterBypassFailure>\n Write Output To Data Store Memory := %<ToDataStoreMemory>
      mask Help:
      | eval('path_lib=fileparts(which(''AEMS_Standard_Library''));');
      | doc_path = [path_lib '\help\AEMS_DEM_COUNTER_BASED_DEBOUNCE_THRSHOLD_DYN.pdf'];
      | eval('open(doc_path)');
      mask Callback eventid:
      | lib_path=gcb;
      | EventID=get_param(lib_path,'eventid');
      | Splitname=regexp(EventID,'_','all');
      | EventID_Name=extractAfter(EventID,EventID(1:Splitname(2)));
      | 
      | Inc_size=strcat('Cnx_dem_pfail_inc_step_',EventID_Name);
      | set_param(lib_path,'DemCounterIncrementStepSize',Inc_size);
      | 
      | Jumpup=strcat('Cbx_dem_jmp_up_act_',EventID_Name);
      | set_param(lib_path,'DemCounterJumpUp',Jumpup);
      | 
      | Jumpup_value=strcat('Cnx_dem_jmp_up_pfail_',EventID_Name);
      | set_param(lib_path,'DemCounterJumpUpValue',Jumpup_value);
      | 
      | Dec_size=strcat('Cnx_dem_ppass_dec_step_',EventID_Name);
      | set_param(lib_path,'DemCounterDecrementStepSize',Dec_size);
      | 
      | Jumpdown=strcat('Cbx_dem_jmp_dwn_act_',EventID_Name);
      | set_param(lib_path,'DemCounterJumpDown',Jumpdown);
      | 
      | Jumpdown_value=strcat('Cnx_dem_jmp_dwn_ppass_',EventID_Name);
      | set_param(lib_path,'DemCounterJumpDownValue',Jumpdown_value);
      | 
      | BypassFailure=strcat('Cbx_dem_byp_fail_',EventID_Name);
      | set_param(lib_path,'DemCounterBypassFailure',BypassFailure);
      | 
      | ToDataStoreMemory = get_param(lib_path,'ToDataStoreMemory');
      | 
      | if strcmpi(ToDataStoreMemory,'on')
      | model_type_pos = strsplit(lib_path,'/');%to split all the layer paths in order to get the runnable path
      | runnable_path = [bdroot '/' model_type_pos{2}];%to get the runnable or AIPCALL path
      | trg_port_name = get_param(find_system(runnable_path,'BlockType','TriggerPort'),'Name');%to get the function call trigger name
      | TaskRate = '';%the raster suffix is stored in the parameter
      | 
      | if ~isempty(trg_port_name)
      |     trg_port_name_spltd = strsplit(trg_port_name{1},'_');%splitting is done in order to get the raster and its type(Sched or Event)
      | 
      |     % checking for rasters of type Sched or Event especially occuring in
      |     % runnables
      |     if ~isempty(regexp(trg_port_name_spltd{1},'^Sched\d+(ms|s)$|^Event+(sync|knock|comc|coml|dcmcb)$','once'))
      |         TaskRate = ['_' regexp(trg_port_name_spltd{1},'\d+(ms|s)$|sync$|knock$|comc$|coml$|dcmcb$','match','once')];
      | 
      |     %checking if the raster is dcmcb and this is applicable only for
      |     %APICALL
      |     elseif ~isempty(regexp([trg_port_name_spltd{1} '_' trg_port_name_spltd{2} '_' ],'^DataServices_DCM_|^RoutineServices_DCM_','once'))||...
      |             ~isempty(regexp(trg_port_name_spltd{1},'^Dcm$','once'))
      |         TaskRate = '_dcmcb';
      | 
      |     %checking if this block is used under the function call trigger
      |     %starting with "Com" and then giving an error message
      |     %this is applicable only for APICALL
      |     elseif ~isempty(regexp(trg_port_name_spltd{1},'^Com$','once'))
      |         msg = sprintf(['\n','The DEM blocks "' Thisblk '" should not be present within APICALLs having function call trigger as "Com"']);
      |         errordlg(msg);
      |         return;
      |     end
      | end
      | DataStoreName = [EventID TaskRate];%the variable name that should be given to DataStoreRead block
      | set_param([lib_path,'/Data Store Write'],'DataStoreName',DataStoreName);
      | else
      |     %do nothing
      | end
      mask Callback Specificchoix:
      | Outputs_From_get_param = get_param(gcb,'Dim_num');
      | Specificchoice_get_param = get_param(gcb,'Specificchoix');
      | maskobj = Simulink.Mask.get(gcbh);
      | maskobj_param = maskobj.Parameters;
      |     if strcmpi(Specificchoice_get_param,'on')
      |        Non=4;
      |         maskobj_param(3).Visible = 'on';
      |         maskobj_param(3).Enabled = 'on';
      |         switch(Outputs_From_get_param)
      |             case '1'
      |                 Non=4;
      |             case '2'
      |                 Non=5;
      |             case '3'
      |                 Non=6;
      |              case '4'
      |                  Non=7;
      |              case '6'
      |                  Non=9;
      |              case '8'
      |                  Non=11;
      |         end
      |     else
      |         maskobj_param(3).Visible = 'off';
      |         maskobj_param(3).Enabled = 'off';
      |         Non=4;
      |     end
      | for i=4:Non
      |     maskobj_param(i).Visible = 'on';
      |     maskobj_param(i).Enabled = 'on';
      | end
      | for i=Non+1:11
      |     maskobj_param(i).Visible = 'off';
      |     maskobj_param(i).Enabled = 'off';
      | end
      | clear maskobj_param;
      | clear maskobj;
      mask TypeOptions Dim_num: 1 | 2 | 3 | 4 | 6 | 8
      mask Callback Dim_num:
      | Outputs_From_get_param = get_param(gcb,'Dim_num');
      | Specificchoice_get_param = get_param(gcb,'Specificchoix');
      | maskobj = Simulink.Mask.get(gcbh);
      | maskobj_param = maskobj.Parameters;
      |     if strcmpi(Specificchoice_get_param,'on')
      |        Non=4;
      |         maskobj_param(3).Visible = 'on';
      |         maskobj_param(3).Enabled = 'on';
      |         switch(Outputs_From_get_param)
      |             case '1'
      |                 Non=4;
      |             case '2'
      |                 Non=5;
      |             case '3'
      |                 Non=6;
      |              case '4'
      |                  Non=7;
      |              case '6'
      |                  Non=9;
      |              case '8'
      |                  Non=11;
      |         end
      |     else
      |         maskobj_param(3).Visible = 'off';
      |         maskobj_param(3).Enabled = 'off';
      |         Non=4;
      |     end
      | for i=4:Non
      |     maskobj_param(i).Visible = 'on';
      |     maskobj_param(i).Enabled = 'on';
      | end
      | for i=Non+1:11
      |     maskobj_param(i).Visible = 'off';
      |     maskobj_param(i).Enabled = 'off';
      | end
      | clear maskobj_param;
      | clear maskobj;
      mask TypeOptions DemDebounceBehavior1: DEM_DEBOUNCE_FREEZE (0) | DEM_DEBOUNCE_RESET (1)
      mask TypeOptions DemDebounceBehavior2: DEM_DEBOUNCE_FREEZE (0) | DEM_DEBOUNCE_RESET (1)
      mask TypeOptions DemDebounceBehavior3: DEM_DEBOUNCE_FREEZE (0) | DEM_DEBOUNCE_RESET (1)
      mask TypeOptions DemDebounceBehavior4: DEM_DEBOUNCE_FREEZE (0) | DEM_DEBOUNCE_RESET (1)
      mask TypeOptions DemDebounceBehavior5: DEM_DEBOUNCE_FREEZE (0) | DEM_DEBOUNCE_RESET (1)
      mask TypeOptions DemDebounceBehavior6: DEM_DEBOUNCE_FREEZE (0) | DEM_DEBOUNCE_RESET (1)
      mask TypeOptions DemDebounceBehavior7: DEM_DEBOUNCE_FREEZE (0) | DEM_DEBOUNCE_RESET (1)
      mask TypeOptions DemDebounceBehavior8: DEM_DEBOUNCE_FREEZE (0) | DEM_DEBOUNCE_RESET (1)
  AEMS_DEM_GET_EVENT_STS : Subsystem  Tag=[LIB]  mask(AEMS_DEM_GET_EVENT_STS){DiagName=EventId_XXXX, LibType=_DGN, FunctionMode=Dysfunctional, Specificchoix=off, Dim_num=1}
      mask prompts: DiagName "Identification of an event:"; LibType "DEM Library type :"; FunctionMode "Function Mode"; Specificchoix "Specific case used only for Nissan cases"; Dim_num "Dimension :"
      mask help:
      | [Get Event Status]
      | - Gets the current extended event status of an event.
      | - "Get Event Status" must be placed in all models including read diagnosis results.
      | - Refer the AUTOSAR Dem_GetEventStatus [SWS_Dem_00195]
      |
      | -OUTPUTS-
      | diag_status_flag: diagnosis status
      |
      | -PARAMETERS-
      | Identification of an event: Enter Identification of an event
      | DEM Library type: Select type of diagnosis result
      |
      | When specific case used only for Nissan cases is checked:
      | Dimension: Select dimension corresponding to diagnosis dimension
      mask init:
      | % EventId = ['Dem_EventId_' DiagName];
      | % eval([char(EventId) '= 0;'])
      | lib_path = gcb;
      | if strcmpi(Specificchoix,'off')
      |    Dim_num='1'; 
      | end
      | %Specify child
      | child_lib = find_system(lib_path,'LookUnderMasks','all','FollowLinks','on','Name','AEMS_DEM_GET_EVENT_STS_D');
      | switch Dim_num
      |     case '1'
      |         if ismember(get_param(child_lib,'MaskType'),{'AEMS_DEM_GET_EVENT_STS_1D'})
      |         else
      |             replace_block(lib_path,'FollowLinks','on','Name','AEMS_DEM_GET_EVENT_STS_D','AEMS_Standard_Library/SUB/AEMS_DEM_GET_EVENT_STS_1D','noprompt');
      |         end
      |     case '2'
      |         if ismember(get_param(child_lib,'MaskType'),{'AEMS_DEM_GET_EVENT_STS_2D'})
      |         else
      |             replace_block(lib_path,'FollowLinks','on','Name','AEMS_DEM_GET_EVENT_STS_D','AEMS_Standard_Library/SUB/AEMS_DEM_GET_EVENT_STS_2D','noprompt');
      |         end
      |     case '8'
      |         if ismember(get_param(child_lib,'MaskType'),{'AEMS_DEM_GET_EVENT_STS_8D'})
      |         else
      |             replace_block(lib_path,'FollowLinks','on','Name','AEMS_DEM_GET_EVENT_STS_D','AEMS_Standard_Library/SUB/AEMS_DEM_GET_EVENT_STS_8D','noprompt');
      |         end
      |     case '9'
      |         if ismember(get_param(child_lib,'MaskType'),{'AEMS_DEM_GET_EVENT_STS_9D'})
      |         else
      |             replace_block(lib_path,'FollowLinks','on','Name','AEMS_DEM_GET_EVENT_STS_D','AEMS_Standard_Library/SUB/AEMS_DEM_GET_EVENT_STS_9D','noprompt');
      |         end
      | end
      | 
      | %Set Diagnosis parameters
      | % set_param([child_lib{:}],'DiagName',char(DiagName));
      | set_param([child_lib{:}],'EventId',char(DiagName));
      | set_param([child_lib{:}],'LibType',char(LibType));
      | set_param([child_lib{:}],'FunctionMode',char(FunctionMode));
      settings: AttributesFormatString=%<MaskType>\nEventId : = %<DiagName>\nDEM Library type : = %<LibType>\nFunction Mode : = %<FunctionMode>\nSpecific case used only for Nissan cases = %<Specificchoix>
      mask Help:
      | eval('path_lib=fileparts(which(''AEMS_Standard_Library''));');
      | doc_path = [path_lib '\help\AEMS_DEM_GET_EVENT_STS.pdf'];
      | eval('open(doc_path)')
      mask TypeOptions LibType: _DGN | _FS(Hold at Key On) | _FS(Reset at Key On) | _NBC | _NGBU | _M7NGBU | _NGREM | _NGMEM | _MIL | _FMILON | _FDGNOK | _MEM | _FLGMEM
      mask TypeOptions FunctionMode: Dysfunctional | From Data Store memory
      mask Callback Specificchoix:
      | maskobj = Simulink.Mask.get(gcbh);
      | maskobj_param = maskobj.Parameters;
      | if strcmp(get(gcbh,'Specificchoix'),'on')
      |     maskobj_param(5).Visible = 'on';
      |     maskobj_param(5).Enabled = 'on';
      | else
      |     maskobj_param(5).Visible = 'off';
      |     maskobj_param(5).Enabled = 'off';
      | end
      | clear maskobj_param;
      | clear maskobj;
      mask TypeOptions Dim_num: 1 | 2 | 8 | 9
      mask Display:
      | dgn_mask = '';
      | 
      | switch LibType
      |     case '_DGN'
      |         dgn_mask = [dgn_mask 'pendingDTC or warningIndicatorRequested\n EventId: ' DiagName '\n Library type: _DGN'];
      |     case '_FS(Hold at Key On)'
      |         dgn_mask = [dgn_mask 'testFailed (Hold at Key On)\n EventId: ' DiagName '\n Library type: _FS'];
      |     case '_FS(Reset at Key On)'
      |         dgn_mask = [dgn_mask 'testFailed (Reset at Key On)\n EventId: ' DiagName '\n Library type: _FS'];
      |     case '_NBC'
      |         dgn_mask = [dgn_mask 'testFailedThisOperationCycle\n EventId: ' DiagName '\n Library type: _NBC'];
      |     case '_NGBU'
      |         dgn_mask = [dgn_mask 'pendingDTC\n EventId: ' DiagName '\n Library type: _NGBU'];
      |     case '_M7NGBU'
      |         dgn_mask = [dgn_mask 'pendingDTC\n EventId: ' DiagName '\n Library type: _M7NGBU'];
      |     case '_NGREM'
      |         dgn_mask = [dgn_mask 'confirmedDTC\n EventId: ' DiagName '\n Library type: _NGREM'];
      |     case '_NGMEM'
      |         dgn_mask = [dgn_mask 'testFailedSinceLastClear\n EventId: ' DiagName '\n Library type: _NGMEM'];
      |     case '_MIL'
      |         dgn_mask = [dgn_mask 'warningIndicatorRequested\n EventId: ' DiagName '\n Library type: _MIL'];
      |     case '_FMILON'
      |         dgn_mask = [dgn_mask 'warningIndicatorRequested\n EventId: ' DiagName '\n Library type: _FMILON'];
      |     case '_FDGNOK'
      |         dgn_mask = [dgn_mask 'TestFailedThisOperationCycle\n EventId: ' DiagName '\n Library type: _FDGNOK'];
      |     case '_MEM'
      |         dgn_mask = [dgn_mask 'TestFailedSinceLastClear\n EventId: ' DiagName '\n Library type: _MEM'];
      |     case '_FLGMEM'
      |         dgn_mask = [dgn_mask 'TestFailedSinceLastClear\n EventId: ' DiagName '\n Library type: _FLGMEM'];
      | end
      | 
      | if strcmpi(Specificchoix,'on')
      |     set(gcbh,'AttributesFormatString','%<MaskType>\nEventId : = %<DiagName>\nDEM Library type : = %<LibType>\nFunction Mode : = %<FunctionMode>\nSpecific case used only for Nissan cases = %<Specificchoix>\nDimension : = %<Dim_num>');
      | else
      |     set(gcbh,'AttributesFormatString','%<MaskType>\nEventId : = %<DiagName>\nDEM Library type : = %<LibType>\nFunction Mode : = %<FunctionMode>\nSpecific case used only for Nissan cases = %<Specificchoix>');
      | end
      | 
      | disp(dgn_mask);
      | plot([5,5,5])
      | plot([6,6,6])
  AEMS_DEM_GET_INDICATOR_STS : Subsystem  Tag=[LIB]  mask(AEMS_DEM_GET_INDICATOR_STS){IndicatorId=0 : IndicatorOff, SimulationMode=0 : Indicator off mode}
      mask prompts: IndicatorId "IndicatorId :"; SimulationMode "Simulation Mode"
      mask help:
      | [Get Indicator Status]
      | - Refer the AUTOSAR Dem_GetIndicatorStatus [SWS_Dem_00205]
      mask init:
      | ThisBlk=gcb;
      | indicator_label = IndicatorId(strfind(IndicatorId,':')+2:length(IndicatorId));
      | indicator_num = IndicatorId(1:strfind(IndicatorId,':')-2);
      | 
      | indicatorid_b = find_system(ThisBlk,'LookUnderMasks','all','FollowLinks','on','Name','IndicatorId_Block');
      | set_param([ThisBlk,'/AEMS_DEM_GETINDICATORSTATUS'],'SimulationMode',char(SimulationMode));
      | set_param([ThisBlk,'/AEMS_DEM_GETINDICATORSTATUS'],'IndicatorId',char(IndicatorId));
      | % % When there is no need for a name in the signal for inputting to AUTOSAR function
      | % set_param([indicatorid_b{:}],'Value',indicator_num);
      | % % ----------
      | 
      | % When a name is required as a signal to input to AUTOSAR function
      | eval([char(indicator_label) ' = ' char(indicator_num) ';']);
      | set_param([indicatorid_b{:}],'Value',char(indicator_label));
      | % ----------
      settings: AttributesFormatString=|
      | %<MaskType>\nIndicatorId = %<IndicatorId>
      | Simulation Mode = %<SimulationMode>
      mask Help:
      | Dem_GetIndicatorStatus [SWS_Dem_00205]
      | Gets the indicator status derived from the event status.
      mask TypeOptions IndicatorId: 0 : IndicatorOff | 1 : DemMILIndicator | 2 : DemRedStopIndicator | 3 : DemAmberWarningIndicator | 4 : DemMessageIndicator1 | 5 : DemMessageIndicator2 | 6 : DemMessageIndicator3 | 7 : DemMessageIndicator4 | 8 : DemMessageIndicator5 | 9 : DemMessageIndicator6 | 10 : DemMessageIndicator7 | 11 : DemMessageIndicator8 | 12 : DemMessageIndicator9 | 13 : DemMessageIndicator10 | 14 : DemMessageIndicator11 | 15 : DemMessageIndicator12 | 16 : DemMessageIndicator13 | 17 : DemMessageIndicator14 | 18 : DemMessageIndicator15 | 19 : DemMessageIndicator16 | 20 : DemMessageIndicator17 | 21 : DemMessageIndicator18 | 22 : DemMessageIndicator19 | 23 : DemMessageIndicator20
      mask TypeOptions SimulationMode: 0 : Indicator off mode | 1 : Indicator continuously on mode | 2 : Indicator blinking mode | 3 : Indicator blinking or continuously on mode | 4 : Indicator slow flashing mode | 5 : Indicator fast flashing mode | 6 : Indicator on-demand mode | 7 : Indicator short mode | From Data Store memory
      mask Display:
      | disp(['Dem_GetIndicatorStatus\n\n\n' IndicatorId]);
      | 
      | port_label('output',1,'indicator_status');
      | 
      | plot([5,5,5])
      | plot([6,6,6])
  AEMS_DEM_READ_DATA_PID01 : Subsystem  Tag=[LIB]  mask(AEMS_DEM_READ_DATA_PID01){}
      mask help:
      | [Read Data PID01]
      | - Refer the AUTOSAR Dem_ReadDataOfPID01 [SWS_Dem01167]
      |
      | Service to report the value of IPD $01 computed by the Dem.
      | API is needed in OBD relevant ECUs only.
      settings: AttributesFormatString=%<MaskType>
      mask Help:
      | eval('path_lib=fileparts(which(''AEMS_Standard_Library''));');
      | doc_path = [path_lib '\help\AEMS_DEM_READ_DATA_PID01.pdf'];
      | eval('open(doc_path)')
      mask Display:
      | disp('Dem_ReadDataOfPID01\n\n');
      | 
      | port_label('output',1,'vpid01');
      | 
      | plot([5,5,5])
      | plot([6,6,6])
  AEMS_DEM_REP_IUMPR : Subsystem  Tag=[LIB]  Description=|  mask(AEMS_DEM_REP_IUMPR){RatioId=Dem_RatioId_XXX, Specificchoix=off, Dim_num=1}
      | !! This Block is Forbidden !!
      | This block is split as two,
      | AEMS_DEM_REP_IUMPR_DEN_RELEASE
      | AEMS_DEM_REP_IUMPR_FAULTDETECT
      mask prompts: RatioId "RatioId :"; Specificchoix "Specific case used only for Nissan cases"; Dim_num "Dimension :"
      mask help:
      | [Dem_RepIUMPRFaultDetect]
      | Service for reporting that faults are possibly found because all conditions are fulfilled.
      |
      | Dimension: Select dimension corresponding to diagnosis dimension
      |
      | RatioId: Automatically filled (No one can edit)
      mask init:
      | % RatioId = ['Dem_RatioId_' DiagName];
      | lib_path = gcb;
      | RatioId = get_param(lib_path,'RatioId');
      | eval([char(RatioId) '= 0;'])
      | 
      | %Specify child
      | child_lib = find_system(lib_path,'LookUnderMasks','all','FollowLinks','on','Name','DEM_REP_IUMPR_D');
      | 
      | if strcmpi(Specificchoix,'off')
      |     Dim_num='1';
      | end
      | 
      | switch Dim_num
      |     case '1'
      |         blk_rep = 'AEMS_DEM_REP_IUMPR_1D';
      |     case '2'
      |         blk_rep = 'AEMS_DEM_REP_IUMPR_2D';
      |     case '8'
      |         blk_rep = 'AEMS_DEM_REP_IUMPR_8D';
      | end
      | if ismember(get_param(child_lib,'MaskType'),{blk_rep})
      | else
      |     replace_block(lib_path,'FollowLinks','on','Name','DEM_REP_IUMPR_D',['AEMS_Standard_Library/SUB/',blk_rep],'noprompt');
      | end
      | 
      | %Set Diagnosis parameters
      | % set_param([child_lib{:}],'DiagName',char(DiagName));
      | set_param([child_lib{:}],'RatioId',char(RatioId));
      settings: AttributesFormatString=%<MaskType>\nRatioId : = %<RatioId>\nSpecific case used only for Nissan cases = %<Specificchoix>
      mask Help:
      | Dem_RepIUMPRFaultDetect [SWS_Dem_00313]
      | Service for reporting that faults are possibly found because all conditions are fulfilled.
      mask Callback RatioId: % set_param(gcb,'RatioId',['Dem_RatioId_' get_param(gcb,'DiagName')]);
      mask Callback Specificchoix:
      | maskobj = Simulink.Mask.get(gcbh);
      | maskobj_param = maskobj.Parameters;
      | if strcmp(get(gcbh,'Specificchoix'),'on')
      |     maskobj_param(3).Visible = 'on';
      |     maskobj_param(3).Enabled = 'on';
      | else
      |     maskobj_param(3).Visible = 'off';
      |     maskobj_param(3).Enabled = 'off';
      | end
      | clear maskobj_param;
      | clear maskobj;
      mask TypeOptions Dim_num: 1 | 2 | 8
      mask Display:
      | port_label('input',1,'denlock_status');
      | port_label('input',2,'faultdetect_trigger');
      | 
      | if strcmpi(Specificchoix,'on')
      |     dgn_mask = [RatioId,'\nDimension : ',Dim_num];
      |     set(gcbh,'AttributesFormatString','%<MaskType>\nRatioId : = %<RatioId>\nSpecific case used only for Nissan cases = %<Specificchoix>\nDimension : = %<Dim_num>');
      | else
      |     dgn_mask = RatioId;
      |     set(gcbh,'AttributesFormatString','%<MaskType>\nRatioId : = %<RatioId>\nSpecific case used only for Nissan cases = %<Specificchoix>');
      | end
      | %disp(dgn_mask);
      | plot([5,5,5])
      | plot([6,6,6])
      | 
      | disp([dgn_mask '\n!! This Block is obsolete and should not be used !!\n use AEMS_DEM_REP_IUMPR_DEN_RELEASE\nand AEMS_DEM_REP_IUMPR_FAULTDETECT instead'])
  AEMS_DEM_REP_IUMPR_DEN_RELEASE : Subsystem  Tag=[LIB]  mask(AEMS_DEM_REP_IUMPR_DEN_RELEASE){RatioId=Dem_RatioId_XXX, Specificchoix=off, Dim_num=1}
      mask prompts: RatioId "RatioId :"; Specificchoix "Specific case used only for Nissan cases"; Dim_num "Dimension :"
      mask help:
      | [Dem_RepIUMPRFaultDetect]
      | Service for reporting that faults are possibly found because all conditions are fulfilled.
      |
      | Dimension:
      | This field is visible only when the Nissan Specific is checked.
      | Select dimension corresponding to diagnosis dimension.
      |
      | RatioId: Automatically filled (It shouldn't be edited)
      mask init:
      | % RatioId = ['Dem_RatioId_' DiagName];
      | lib_path = gcb;
      | RatioId = get_param(lib_path,'RatioId');
      | eval([char(RatioId) '= 0;'])
      | 
      | %Specify child
      | %child_lib = find_system(lib_path,'LookUnderMasks','all','FollowLinks','on','Name','DEM_REP_IUMPR_DEN_RELEASE_D');
      | child_lib = [lib_path,'/DEM_REP_IUMPR_DEN_RELEASE_D'];
      | 
      | if strcmpi(Specificchoix,'off')
      |     Dim_num='1';
      | end
      | 
      | switch Dim_num
      |     case '1'
      |         blk_rep = 'AEMS_DEM_REP_IUMPR_DEN_RELEASE_1D';
      |     case '2'
      |         blk_rep = 'AEMS_DEM_REP_IUMPR_DEN_RELEASE_2D';
      |     case '8'
      |         blk_rep = 'AEMS_DEM_REP_IUMPR_DEN_RELEASE_8D';
      | end
      | 
      | if ~strcmp(get_param(child_lib,'MaskType'),blk_rep)
      |     replace_block(lib_path,'FollowLinks','on','Name','DEM_REP_IUMPR_DEN_RELEASE_D',['AEMS_Standard_Library/SUB/',blk_rep],'noprompt');
      | end
      | 
      | %Set Diagnosis parameters
      | % set_param([child_lib{:}],'DiagName',char(DiagName));
      | set_param(child_lib,'RatioId',RatioId);
      settings: AttributesFormatString=%<MaskType>\nRatioId : = %<RatioId>\nSpecific case used only for Nissan cases = %<Specificchoix>
      mask Help:
      | eval('path_lib=fileparts(which(''AEMS_Standard_Library''));');
      | doc_path = [path_lib '\help\AEMS_DEM_REP_IUMPR_DEN_RELEASE.pdf'];
      | eval('open(doc_path)')
      | 
      | Dem_RepIUMPRFaultDetect [SWS_Dem_00313]
      | Service for reporting that faults are possibly found because all conditions are fulfilled.
      mask Callback RatioId: % set_param(gcb,'RatioId',['Dem_RatioId_' get_param(gcb,'DiagName')]);
      mask Callback Specificchoix:
      | maskobj = Simulink.Mask.get(gcbh);
      | maskobj_param = maskobj.Parameters;
      | if strcmp(get(gcbh,'Specificchoix'),'on')
      |     maskobj_param(3).Visible = 'on';
      |     maskobj_param(3).Enabled = 'on';
      | else
      |     maskobj_param(3).Visible = 'off';
      |     maskobj_param(3).Enabled = 'off';
      | end
      | clear maskobj_param;
      | clear maskobj;
      mask TypeOptions Dim_num: 1 | 2 | 8
      mask Display:
      | port_label('input',1,'denlock_status');
      | 
      | if strcmpi(Specificchoix,'on')
      |     dgn_mask = [RatioId,'\nDimension : ',Dim_num];
      |     set(gcbh,'AttributesFormatString','%<MaskType>\nRatioId : = %<RatioId>\nSpecific case used only for Nissan cases = %<Specificchoix>\nDimension : = %<Dim_num>');
      | else
      |     dgn_mask = RatioId;
      |     set(gcbh,'AttributesFormatString','%<MaskType>\nRatioId : = %<RatioId>\nSpecific case used only for Nissan cases = %<Specificchoix>');
      | end
      | disp(dgn_mask);
      | plot([5,5,5])
      | plot([6,6,6])
  AEMS_DEM_REP_IUMPR_FAULTDETECT : Subsystem  Tag=[LIB]  mask(AEMS_DEM_REP_IUMPR_FAULTDETECT){RatioId=Dem_RatioId_XXX, Specificchoix=off, Dim_num=1}
      mask prompts: RatioId "RatioId :"; Specificchoix "Specific case used only for Nissan cases"; Dim_num "Dimension :"
      mask help:
      | [Dem_RepIUMPRFaultDetect]
      | Service for reporting that faults are possibly found because all conditions are fulfilled.
      |
      | Dimension:
      | This field is visible only when the Nissan Specific is checked.
      | Select dimension corresponding to diagnosis dimension.
      |
      | RatioId: Automatically filled (It shouldn't be edited)
      mask init:
      | % RatioId = ['Dem_RatioId_' DiagName];
      | lib_path = gcb;
      | RatioId = get_param(lib_path,'RatioId');
      | eval([char(RatioId) '= 0;'])
      | 
      | %Specify child
      | %child_lib = find_system(lib_path,'LookUnderMasks','all','FollowLinks','on','Name','DEM_REP_IUMPR_DEN_RELEASE_D');
      | child_lib = [lib_path,'/DEM_REP_IUMPR_FAULTDETECT_D'];
      | 
      | if strcmpi(Specificchoix,'off')
      |     Dim_num='1';
      | end
      | 
      | switch Dim_num
      |     case '1'
      |         blk_rep = 'AEMS_DEM_REP_IUMPR_FAULTDETECT_1D';
      |     case '2'
      |         blk_rep = 'AEMS_DEM_REP_IUMPR_FAULTDETECT_2D';
      |     case '8'
      |         blk_rep = 'AEMS_DEM_REP_IUMPR_FAULTDETECT_8D';
      | end
      | if ~strcmp(get_param(child_lib,'MaskType'),blk_rep)
      |     replace_block(lib_path,'FollowLinks','on','Name','DEM_REP_IUMPR_FAULTDETECT_D',['AEMS_Standard_Library/SUB/',blk_rep],'noprompt');
      | end
      | 
      | %Set Diagnosis parameters
      | % set_param([child_lib{:}],'DiagName',char(DiagName));
      | set_param(child_lib,'RatioId',RatioId);
      settings: AttributesFormatString=%<MaskType>\nRatioId : = %<RatioId>\nSpecific case used only for Nissan cases = %<Specificchoix>
      mask Help:
      | eval('path_lib=fileparts(which(''AEMS_Standard_Library''));');
      | doc_path = [path_lib '\help\AEMS_DEM_REP_IUMPR_FAULTDETECT.pdf'];
      | eval('open(doc_path)')
      | 
      | Dem_RepIUMPRFaultDetect [SWS_Dem_00313]
      | Service for reporting that faults are possibly found because all conditions are fulfilled.
      mask Callback RatioId: % set_param(gcb,'RatioId',['Dem_RatioId_' get_param(gcb,'DiagName')]);
      mask Callback Specificchoix:
      | maskobj = Simulink.Mask.get(gcbh);
      | maskobj_param = maskobj.Parameters;
      | if strcmp(get(gcbh,'Specificchoix'),'on')
      |     maskobj_param(3).Visible = 'on';
      |     maskobj_param(3).Enabled = 'on';
      | else
      |     maskobj_param(3).Visible = 'off';
      |     maskobj_param(3).Enabled = 'off';
      | end
      | clear maskobj_param;
      | clear maskobj;
      mask TypeOptions Dim_num: 1 | 2 | 8
      mask Display:
      | port_label('input',1,'faultdetect_trigger');
      | 
      | if strcmpi(Specificchoix,'on')
      |     dgn_mask = [RatioId,'\nDimension : ',Dim_num];
      |     set(gcbh,'AttributesFormatString','%<MaskType>\nRatioId : = %<RatioId>\nSpecific case used only for Nissan cases = %<Specificchoix>\nDimension : = %<Dim_num>');
      | else
      |     dgn_mask = RatioId;
      |     set(gcbh,'AttributesFormatString','%<MaskType>\nRatioId : = %<RatioId>\nSpecific case used only for Nissan cases = %<Specificchoix>');
      | end
      | disp(dgn_mask);
      | plot([5,5,5])
      | plot([6,6,6])
  AEMS_DEM_SET_DTR : Subsystem  Tag=[LIB]  mask(AEMS_DEM_SET_DTR){EventId=Dem_DtrId_XXX, Specificchoix=off, Dim_num=1, conv_type=0x24, unit=1 per bit, resol=1, dlim=0, ulim=65535}
      mask prompts: EventId "DTR Id :"; Specificchoix "Specific case used only for Nissan cases"; Dim_num "Dimension :"; conv_type "Conversion Type"; unit "Resolution and Unit :"; resol "Resolution :"; dlim "Lower Limit :"; ulim "Upper Limit :"
      mask help:
      | Reports a DTR result with lower and upper limit. The internal eventstatus serves
      | as master whether the DTR values are fowareded or ignored,
      | also taking the DTRUpdateKind into account.
      |
      | Conversion Type : Each number has different Resolution, Upper/Lower Limit.
      |                     *Only "0x24" and "0x2B" have data type of "Uint". Others are set to "Single".
      mask init:
      | EventId = get_param(gcb,'EventId');
      | % EventId = ['Dem_DtrId_' DtrId];
      | eval([char(EventId) '= 0;']);
      | % eval([char(Ctrlval) '= 0;']);
      | 
      | lib_path = gcb;
      | child_lib = find_system(lib_path,'LookUnderMasks','all','FollowLinks','on','Name','DEM_SET_DTR_D');
      | if strcmpi(Specificchoix,'off')
      |     Dim_num='1';
      | end
      | switch Dim_num
      |     case '1'
      |         dim_block = 'AEMS_DEM_SET_DTR_1D';
      |     case '2'
      |         dim_block = 'AEMS_DEM_SET_DTR_2D';
      |     case '8'
      |         dim_block = 'AEMS_DEM_SET_DTR_8D';
      |     case '9'
      |         conv_type = '0x24';
      |         dim_block = 'AEMS_DEM_SET_DTR_9D';
      | end
      | 
      | if strcmp(conv_type,'0x2B') || strcmp(conv_type,'0x24')
      |     dim_block_2 = [dim_block,'U'];
      | else
      |     dim_block_2 = [dim_block,'S'];
      | end
      | rep_block = ['AEMS_Standard_Library/SUB/',dim_block_2];
      | if ismember(get_param(child_lib,'MaskType'),{dim_block_2})
      | else
      |     replace_block(lib_path,'FollowLinks','on','Name','DEM_SET_DTR_D',(rep_block),'noprompt');
      | end
      | 
      | switch conv_type
      |     case '0x01'
      |         resol = '1';
      |         ulim = '65535';
      |         dlim = '0';
      |     case '0x02'
      |         resol = '0.1';
      |         ulim = '6553.5';
      |         dlim = '0';
      |     case '0x03'
      |         resol = '0.01';
      |         ulim = '655.35';
      |         dlim = '0';
      |     case '0x04'
      |         resol = '0.001';
      |         ulim = '65.535';
      |         dlim = '0';
      |     case '0x05'
      |         resol = '0.000030517578';
      |         ulim = '1.99996947423';
      |         dlim = '0';
      |     case '0x06'
      |         resol = '0.000305';
      |         ulim = '19.988175';
      |         dlim = '0';
      |     case '0x07'
      |         resol = '0.25';
      |         ulim = '16383.75';
      |         dlim = '0';
      |     case '0x08'
      |         resol = '0.01';
      |         ulim = '655.35';
      |         dlim = '0';
      |     case '0x09'
      |         resol = '1';
      |         ulim = '65535';
      |         dlim = '0';
      |     case '0x0A'
      |         resol = '0.1220703125';
      |         ulim = '7999.8779296875';
      |         dlim = '0';
      |     case '0x0B'
      |         resol = '.001';
      |         ulim = '65.535';
      |         dlim = '0';
      |     case '0x0C'
      |         resol = '.01';
      |         ulim = '655.35';
      |         dlim = '0';
      |     case '0x0D'
      |         resol = '0.00390625';
      |         ulim = '255.99609375';
      |         dlim = '0';
      |     case '0x0E'
      |         resol = '.001';
      |         ulim = '65.535';
      |         dlim = '0';
      |     case '0x0F'
      |         resol = '.01';
      |         ulim = '655.35';
      |         dlim = '0';
      |     case '0x10'
      |         resol = '1';
      |         ulim = '65535';
      |         dlim = '0';
      |     case '0x11'
      |         resol = '100';
      |         ulim = '6553500';
      |         dlim = '0';
      |     case '0x12'
      |         resol = '1';
      |         ulim = '65535';
      |         dlim = '0';
      |     case '0x13'
      |         resol = '1';
      |         ulim = '65535';
      |         dlim = '0';
      |     case '0x14'
      |         resol = '1';
      |         ulim = '65535';
      |         dlim = '0';
      |     case '0x15'
      |         resol = '1';
      |         ulim = '65535';
      |         dlim = '0';
      |     case '0x16'
      |         resol = '0.1';
      |         ulim = '6513.5';
      |         dlim = '-40';
      |     case '0x17'
      |         resol = '0.01';
      |         ulim = '655.35';
      |         dlim = '0';
      |     case '0x18'
      |         resol = '0.0117';
      |         ulim = '766.7595';
      |         dlim = '0';
      |     case '0x19'
      |         resol = '0.079';
      |         ulim = '5177.265';
      |         dlim = '0';
      |     case '0x1A'
      |         resol = '1';
      |         ulim = '65535';
      |         dlim = '0';
      |     case '0x1B'
      |         resol = '10';
      |         ulim = '655350';
      |         dlim = '0';
      |     case '0x1C'
      |         resol = '0.01';
      |         ulim = '655.35';
      |         dlim = '0';
      |     case '0x1D'
      |         resol = '0.5';
      |         ulim = '32767.5';
      |         dlim = '0';
      |     case '0x1E'
      |         resol = '0.000030517578';
      |         ulim = '1.99996947423';
      |         dlim = '0';
      |     case '0x1F'
      |         resol = '0.05';
      |         ulim = '3276.75';
      |         dlim = '0';
      |     case '0x20'
      |         resol = '0.00390625';
      |         ulim = '255.99609375';
      |         dlim = '0';
      |     case '0x21'
      |         resol = '1';
      |         ulim = '65535';
      |         dlim = '0';
      |     case '0x22'
      |         resol = '1';
      |         ulim = '65535';
      |         dlim = '0';
      |     case '0x23'
      |         resol = '1';
      |         ulim = '65535';
      |         dlim = '0';
      |     case '0x25'
      |         resol = '1';
      |         ulim = '65535';
      |         dlim = '0';
      |     case '0x26'
      |         resol = '0.1';
      |         ulim = '6553.5';
      |         dlim = '0';
      |     case '0x27'
      |         resol = '0.01';
      |         ulim = '655.35';
      |         dlim = '0';
      |     case '0x28'
      |         resol = '1';
      |         ulim = '65535';
      |         dlim = '0';
      |     case '0x29'
      |         resol = '0.25';
      |         ulim = '16383.75';
      |         dlim = '0';
      |     case '0x2A'
      |         resol = '.001';
      |         ulim = '65.535';
      |         dlim = '0';
      |     case '0x2C'
      |         resol = '.01';
      |         ulim = '655.35';
      |         dlim = '0';
      |     case '0x2D'
      |         resol = '.01';
      |         ulim = '655.35';
      |         dlim = '0';
      |     case '0x2E'
      |         resol = '1';
      |         ulim = '1';
      |         dlim = '0';
      |     case '0x2F'
      |         resol = '.01';
      |         ulim = '655.35';
      |         dlim = '0';
      |     case '0x30'
      |         resol = '0.001526';
      |         ulim = '100.00641';
      |         dlim = '0';
      |     case '0x31'
      |         resol = '.001';
      |         ulim = '65.535';
      |         dlim = '0';
      |     case '0x32'
      |         resol = '0.00003051757813';
      |         ulim = '1.99996948274955';
      |         dlim = '0';
      |     case '0x33'
      |         resol = '0.000244140625';
      |         ulim = '15.999755859375';
      |         dlim = '0';
      |     case '0x34'
      |         resol = '1';
      |         ulim = '65535';
      |         dlim = '0';
      |     case '0x35'
      |         resol = '10';
      |         ulim = '655350';
      |         dlim = '0';
      |     case '0x36'
      |         resol = '0.01';
      |         ulim = '655.35';
      |         dlim = '0';
      |     case '0x37'
      |         resol = '0.1';
      |         ulim = '6553.5';
      |         dlim = '0';
      |     case '0x38'
      |         resol = '1';
      |         ulim = '65535';
      |         dlim = '0';
      |     case '0x39'
      |         resol = '.01';
      |         ulim = '655.35';
      |         dlim = '0';
      |     case '0x3A'
      |         resol = '0.001';
      |         ulim = '65.535';
      |         dlim = '0';
      |     case '0x3B'
      |         resol = '0.0001';
      |         ulim = '6.5535';
      |         dlim = '0';
      |     case '0x3C'
      |         resol = '0.1';
      |         ulim = '6553.5';
      |         dlim = '0';
      |     case '0x3D'
      |         resol = '.01';
      |         ulim = '655.35';
      |         dlim = '0';
      |     case '0x3E'
      |         resol = '0.00006103516';
      |         ulim = '3.9999392106';
      |         dlim = '0';
      |     case '0x3F'
      |         resol = '0.01';
      |         ulim = '655.35';
      |         dlim = '0';
      |     case '0x40'
      |         resol = '1';
      |         ulim = '65535';
      |         dlim = '0';
      |     case '0x41'
      |         resol = '0.01';
      |         ulim = '655.35';
      |         dlim = '0';
      |     case '0x42'
      |         resol = '0.1';
      |         ulim = '6553.5';
      |         dlim = '0';
      |     case '0x43'
      |         resol = '0.000244140625';
      |         ulim = '15.999755859375';
      |         dlim = '0';
      |     case '0x44'
      |         resol = '1';
      |         ulim = '65535';
      |         dlim = '0';
      |     case '0x81'
      |         resol = '1';
      |         ulim = '32767';
      |         dlim = '-32768';
      |     case '0x82'
      |         resol = '0.1';
      |         ulim = '3276.7';
      |         dlim = '-3276.8';
      |     case '0x83'
      |         resol = '0.01';
      |         ulim = '327.67';
      |         dlim = '-327.68';
      |     case '0x84'
      |         resol = '0.001';
      |         ulim = '32.767';
      |         dlim = '-32.768';
      |     case '0x85'
      |         resol = '0.000030517578';
      |         ulim = '0.999969478326';
      |         dlim = '-0.999999995904';
      |     case '0x86'
      |         resol = '0.000305';
      |         ulim = '9.993935';
      |         dlim = '-9.99424';
      |     case '0x87'
      |         resol = '1';
      |         ulim = '32767';
      |         dlim = '-32768';
      |     case '0x8A'
      |         resol = '0.1220703125';
      |         ulim = '3999.8779296875';
      |         dlim = '-4000';
      |     case '0x8B'
      |         resol = '0.001';
      |         ulim = '32.767';
      |         dlim = '-32.768';
      |     case '0x8C'
      |         resol = '0.01';
      |         ulim = '327.67';
      |         dlim = '-327.68';
      |     case '0x8D'
      |         resol = '0.00390625';
      |         ulim = '127.99609375';
      |         dlim = '-128';
      |     case '0x8E'
      |         resol = '0.001';
      |         ulim = '32.767';
      |         dlim = '-32.768';
      |     case '0x8F'
      |         resol = '1';
      |         ulim = '32767';
      |         dlim = '-32768';
      |     case '0x90'
      |         resol = '1';
      |         ulim = '32767';
      |         dlim = '-32768';
      |     case '0x91'
      |         resol = '0.1';
      |         ulim = '3276.7';
      |         dlim = '-3276.8';
      |     case '0x92'
      |         resol = '0.1';
      |         ulim = '3276.7';
      |         dlim = '-3276.8';
      |     case '0x96'
      |         resol = '0.1';
      |         ulim = '3276.7';
      |         dlim = '-3276.8';
      |     case '0x97'
      |         resol = '0.01';
      |         ulim = '327.67';
      |         dlim = '-327.68';
      |     case '0x98'
      |         resol = '1';
      |         ulim = '32767';
      |         dlim = '-32768';
      |     case '0x99'
      |         resol = '0.1';
      |         ulim = '3276.7';
      |         dlim = '-3276.8';
      |     case '0x9C'
      |         resol = '0.01';
      |         ulim = '327.67';
      |         dlim = '-327.68';
      |     case '0x9D'
      |         resol = '0.5';
      |         ulim = '16383.5';
      |         dlim = '-16384';
      |     case '0xA8'
      |         resol = '1';
      |         ulim = '32767';
      |         dlim = '-32768';
      |     case '0xA9'
      |         resol = '0.25';
      |         ulim = '8191.75';
      |         dlim = '-8192';
      |     case '0xAD'
      |         resol = '0.01';
      |         ulim = '327.67';
      |         dlim = '-327.68';
      |     case '0xAE'
      |         resol = '0.1';
      |         ulim = '3276.7';
      |         dlim = '-3276.8';
      |     case '0xAF'
      |         resol = '0.01';
      |         ulim = '327.67';
      |         dlim = '-327.68';
      |     case '0xB0'
      |         resol = '0.003052';
      |         ulim = '100.004884';
      |         dlim = '-100.007936';
      |     case '0xB1'
      |         resol = '2';
      |         ulim = '65534';
      |         dlim = '-65536';
      |     case '0xFA'
      |         resol = '20';
      |         ulim = '655340';
      |         dlim = '-655360';
      |     case '0xFB'
      |         resol = '10';
      |         ulim = '327670';
      |         dlim = '-327680';
      |     case '0xFC'
      |         resol = '0.01';
      |         ulim = '327.67';
      |         dlim = '-327.68';
      |     case '0xFD'
      |         resol = '0.001';
      |         ulim = '32.767';
      |         dlim = '-32.768';
      |     case '0xFE'
      |         resol = '0.25';
      |         ulim = '8191.75';
      |         dlim = '-8192';
      |     case '0x2B'
      |         resol = '1';
      |         ulim = '65535';
      |         dlim = '0';
      |     case '0x24'
      |         resol = '1';
      |         ulim = '65535';
      |         dlim = '0';
      | end
      | 
      | set_param([child_lib{:}],'conv_type',char(conv_type));
      | % set_param([child_lib{:}],'DtrId',char(DtrId));
      | % set_param([child_lib{:}],'Ctrlval',char(Ctrlval));
      | set_param([child_lib{:}],'EventId',char(EventId));
      | set_param([child_lib{:}],'resol',char(resol));
      | set_param([child_lib{:}],'ulim',char(ulim));
      | set_param([child_lib{:}],'dlim',char(dlim));
      settings: AttributesFormatString=%<MaskType>\nDTR Id : = %<EventId>\nSpecific case used only for Nissan cases = %<Specificchoix>\nConversion Type = %<conv_type>\nResolution and Unit : = %<unit>\nLower Limit : = %<dlim>\nUpper Limit : = %<ulim>
      mask Help:
      | eval('path_lib=fileparts(which(''AEMS_Standard_Library''));');
      | doc_path = [path_lib '\help\AEMS_DEM_SET_DTR.pdf'];
      | eval('open(doc_path)')
      mask Callback EventId: % set_param(gcb,'EventId',['Dem_DtrId_' get_param(gcb,'DtrId')]);
      mask Callback Specificchoix:
      | maskobj = Simulink.Mask.get(gcbh);
      | maskobj_param = maskobj.Parameters;
      | if strcmp(get(gcbh,'Specificchoix'),'on')
      |     maskobj_param(3).Visible = 'on';
      |     maskobj_param(3).Enabled = 'on';
      | else
      |     maskobj_param(3).Visible = 'off';
      |     maskobj_param(3).Enabled = 'off';
      | end
      | clear maskobj;
      | clear maskobj_param;
      mask TypeOptions Dim_num: 1 | 2 | 8 | 9
      mask Callback Dim_num:
      | if ismember(get_param(gcb,'Dim_num'),'9');
      |         set_param(gcb,'conv_type','0x24');
      |         set_param(gcb,'resol','1');
      |         set_param(gcb,'ulim','65535');
      |         set_param(gcb,'dlim','0');
      |         set_param(gcb,'unit','1 per bit');
      |     set_param(gcb,'MaskEnableString','on,on,on,off,off,off,off,off');
      | else
      |     set_param(gcb,'MaskEnableString','on,on,on,on,off,off,off,off');
      | end
      mask TypeOptions conv_type: 0x01 | 0x02 | 0x03 | 0x04 | 0x05 | 0x06 | 0x07 | 0x08 | 0x09 | 0x0A | 0x0B | 0x0C | 0x0D | 0x0E | 0x0F | 0x10 | 0x11 | 0x12 | 0x13 | 0x14 | 0x15 | 0x16 | 0x17 | 0x18 | 0x19 | 0x1A | 0x1B | 0x1C | 0x1D | 0x1E | 0x1F | 0x20 | 0x21 | 0x22 | 0x23 | 0x24 | 0x25 | 0x26 | 0x27 | 0x28 | 0x29 | 0x2A | 0x2B | 0x2C | 0x2D | 0x2E | 0x2F | 0x30 | 0x31 | 0x32 | 0x33 | 0x34 | 0x35 | 0x36 | 0x37 | 0x38 | 0x39 | 0x3A | 0x3B | 0x3C | 0x3D | 0x3E | 0x3F | 0x40 | 0x41 | 0x42 | 0x43 | 0x44 | 0x81 | 0x82 | 0x83 | 0x84 | 0x85 | 0x86 | 0x87 | 0x8A | 0x8B | 0x8C | 0x8D | 0x8E | 0x8F | 0x90 | 0x91 | 0x92 | 0x96 | 0x97 | 0x98 | 0x99 | 0x9C | 0x9D | 0xA8 | 0xA9 | 0xAD | 0xAE | 0xAF | 0xB0 | 0xB1 | 0xFA | 0xFB | 0xFC | 0xFD | 0xFE
      mask Callback conv_type:
      | contype_case = get_param(gcb, 'conv_type');
      | switch contype_case
      |     case '0x01'
      |         set_param(gcb, 'resol', '1');
      |         set_param(gcb,'ulim','65535');
      |         set_param(gcb,'dlim','0');
      |         set_param(gcb,'unit','1 per bit');
      |     case '0x02'
      |         set_param(gcb, 'resol', '0.1');
      |         set_param(gcb,'ulim','6553.5');
      |         set_param(gcb,'dlim','0');
      |         set_param(gcb,'unit','0.1 per bit');
      |     case '0x03'
      |         set_param(gcb, 'resol', '0.01');
      |         set_param(gcb,'ulim','655.35');
      |         set_param(gcb,'dlim','0');
      |         set_param(gcb,'unit',' 0.01 per bit');
      |     case '0x04'
      |         set_param(gcb, 'resol', '0.001');
      |         set_param(gcb,'ulim','65.535');
      |         set_param(gcb,'dlim','0');
      |         set_param(gcb,'unit',' 0.001 per bit');
      |     case '0x05'
      |         set_param(gcb, 'resol', '0.000030517578');
      |         set_param(gcb,'ulim','1.99996947423');
      |         set_param(gcb,'dlim','0');
      |         set_param(gcb,'unit','0.000030517578 per bit');
      |     case '0x06'
      |         set_param(gcb, 'resol', '0.000305');
      |         set_param(gcb,'ulim','19.988175');
      |         set_param(gcb,'dlim','0');
      |         set_param(gcb,'unit','0.000305 per bit');
      |     case '0x07'
      |         set_param(gcb, 'resol', '0.25');
      |         set_param(gcb,'ulim','16383.75');
      |         set_param(gcb,'dlim','0');
      |         set_param(gcb,'unit','0.25  rpm per bit');
      |     case '0x08'
      |         set_param(gcb, 'resol', '0.01');
      |         set_param(gcb,'ulim','655.35');
      |         set_param(gcb,'dlim','0');
      |         set_param(gcb,'unit','0.01 km/h per bit');
      |     case '0x09'
      |         set_param(gcb, 'resol', '1');
      |         set_param(gcb,'ulim','65535');
      |         set_param(gcb,'dlim','0');
      |         set_param(gcb,'unit','1 km/h per bit');
      |     case '0x0A'
      |         set_param(gcb, 'resol', '0.1220703125');
      |         set_param(gcb,'ulim','7999.8779296875');
      |         set_param(gcb,'dlim','0');
      |         set_param(gcb,'unit','0.1220703125 mV per bit');
      |     case '0x0B'
      |         set_param(gcb, 'resol', '.001');
      |         set_param(gcb,'ulim','65.535');
      |         set_param(gcb,'dlim','0');
      |         set_param(gcb,'unit','0.001 V per bit');
      |     case '0x0C'
      |         set_param(gcb, 'resol', '.01');
      |         set_param(gcb,'ulim','655.35');
      |         set_param(gcb,'dlim','0');
      |         set_param(gcb,'unit','0.01 V per bit');
      |     case '0x0D'
      |         set_param(gcb, 'resol', '0.00390625');
      |         set_param(gcb,'ulim','255.99609375');
      |         set_param(gcb,'dlim','0');
      |         set_param(gcb,'unit','0.00390625 mA per bit');
      |     case '0x0E'
      |         set_param(gcb, 'resol', '.001');
      |         set_param(gcb,'ulim','65.535');
      |         set_param(gcb,'dlim','0');
      |         set_param(gcb,'unit','0.001 A per bit');
      |     case '0x0F'
      |         set_param(gcb, 'resol', '.01');
      |         set_param(gcb,'ulim','655.35');
      |         set_param(gcb,'dlim','0');
      |         set_param(gcb,'unit','0.01 A per bit');
      |     case '0x10'
      |         set_param(gcb, 'resol', '1');
      |         set_param(gcb,'ulim','65535');
      |         set_param(gcb,'dlim','0');
      |         set_param(gcb,'unit','1 ms per bit');
      |     case '0x11'
      |         set_param(gcb, 'resol', '100');
      |         set_param(gcb,'ulim','6553500');
      |         set_param(gcb,'dlim','0');
      |         set_param(gcb,'unit','100 ms per bit');
      |     case '0x12'
      |         set_param(gcb, 'resol', '1');
      |         set_param(gcb,'ulim','65535');
      |         set_param(gcb,'dlim','0');
      |         set_param(gcb,'unit','1 s per bit');
      |     case '0x13'
      |         set_param(gcb, 'resol', '1');
      |         set_param(gcb,'ulim','65535');
      |         set_param(gcb,'dlim','0');
      |         set_param(gcb,'unit','1 mOhm per bit');
      |     case '0x14'
      |         set_param(gcb, 'resol', '1');
      |         set_param(gcb,'ulim','65535');
      |         set_param(gcb,'dlim','0');
      |         set_param(gcb,'unit','1 Ohm per bit');
      |     case '0x15'
      |         set_param(gcb, 'resol', '1');
      |         set_param(gcb,'ulim','65535');
      |         set_param(gcb,'dlim','0');
      |         set_param(gcb,'unit','1 kOhm per bit');
      |     case '0x16'
      |         set_param(gcb, 'resol', '0.1');
      |         set_param(gcb,'ulim','6513.5');
      |         set_param(gcb,'dlim','-40');
      |         set_param(gcb,'unit','0.1 oC per bit - 40oC');
      |     case '0x17'
      |         set_param(gcb, 'resol', '0.01');
      |         set_param(gcb,'ulim','655.35');
      |         set_param(gcb,'dlim','0');
      |         set_param(gcb,'unit','0.01 kPa per bit');
      |     case '0x18'
      |         set_param(gcb, 'resol', '0.0117');
      |         set_param(gcb,'ulim','766.7595');
      |         set_param(gcb,'dlim','0');
      |         set_param(gcb,'unit','0.0117 kPa per bit');
      |     case '0x19'
      |         set_param(gcb, 'resol', '0.079');
      |         set_param(gcb,'ulim','5177.265');
      |         set_param(gcb,'dlim','0');
      |         set_param(gcb,'unit','0.079 kPa per bit');
      |     case '0x1A'
      |         set_param(gcb, 'resol', '1');
      |         set_param(gcb,'ulim','65535');
      |         set_param(gcb,'dlim','0');
      |         set_param(gcb,'unit','1 kPa per bit');
      |     case '0x1B'
      |         set_param(gcb, 'resol', '10');
      |         set_param(gcb,'ulim','655350');
      |         set_param(gcb,'dlim','0');
      |         set_param(gcb,'unit','10 kPa per bit');
      |     case '0x1C'
      |         set_param(gcb, 'resol', '0.01');
      |         set_param(gcb,'ulim','655.35');
      |         set_param(gcb,'dlim','0');
      |         set_param(gcb,'unit','0.01 o per bit');
      |     case '0x1D'
      |         set_param(gcb, 'resol', '0.5');
      |         set_param(gcb,'ulim','32767.5');
      |         set_param(gcb,'dlim','0');
      |         set_param(gcb,'unit','0.5 o per bit');
      |     case '0x1E'
      |         set_param(gcb, 'resol', '0.000030517578');
      |         set_param(gcb,'ulim','1.99996947423');
      |         set_param(gcb,'dlim','0');
      |         set_param(gcb,'unit','0.000030517578 per bit');
      |     case '0x1F'
      |         set_param(gcb, 'resol', '0.05');
      |         set_param(gcb,'ulim','3276.75');
      |         set_param(gcb,'dlim','0');
      |         set_param(gcb,'unit','0.05 per bit');
      |     case '0x20'
      |         set_param(gcb, 'resol', '0.00390625');
      |         set_param(gcb,'ulim','255.99609375');
      |         set_param(gcb,'dlim','0');
      |         set_param(gcb,'unit','0.00390625 per bit');
      |     case '0x21'
      |         set_param(gcb, 'resol', '1');
      |         set_param(gcb,'ulim','65535');
      |         set_param(gcb,'dlim','0');
      |         set_param(gcb,'unit','1 mHz per bit');
      |     case '0x22'
      |         set_param(gcb, 'resol', '1');
      |         set_param(gcb,'ulim','65535');
      |         set_param(gcb,'dlim','0');
      |         set_param(gcb,'unit','1 Hz per bit');
      |     case '0x23'
      |         set_param(gcb, 'resol', '1');
      |         set_param(gcb,'ulim','65535');
      |         set_param(gcb,'dlim','0');
      |         set_param(gcb,'unit','1 kHz per bit');
      |     case '0x24'
      |         set_param(gcb, 'resol', '1');
      |         set_param(gcb,'ulim','65535');
      |         set_param(gcb,'dlim','0');
      |         set_param(gcb,'unit','1 per bit');
      |     case '0x25'
      |         set_param(gcb, 'resol', '1');
      |         set_param(gcb,'ulim','65535');
      |         set_param(gcb,'dlim','0');
      |         set_param(gcb,'unit','1 km per bit');
      |     case '0x26'
      |         set_param(gcb, 'resol', '0.1');
      |         set_param(gcb,'ulim','6553.5');
      |         set_param(gcb,'dlim','0');
      |         set_param(gcb,'unit','0.1 mV/ms per bit');
      |     case '0x27'
      |         set_param(gcb, 'resol', '0.01');
      |         set_param(gcb,'ulim','655.35');
      |         set_param(gcb,'dlim','0');
      |         set_param(gcb,'unit','0.01 g/s per bit');
      |     case '0x28'
      |         set_param(gcb, 'resol', '1');
      |         set_param(gcb,'ulim','65535');
      |         set_param(gcb,'dlim','0');
      |         set_param(gcb,'unit','1 g/s per bit');
      |     case '0x29'
      |         set_param(gcb, 'resol', '0.25');
      |         set_param(gcb,'ulim','16383.75');
      |         set_param(gcb,'dlim','0');
      |         set_param(gcb,'unit','0.25 Pa/s per bit');
      |     case '0x2A'
      |         set_param(gcb, 'resol', '.001');
      |         set_param(gcb,'ulim','65.535');
      |         set_param(gcb,'dlim','0');
      |         set_param(gcb,'unit','0.001 kg/h per bit');
      |     case '0x2B'
      |         set_param(gcb, 'resol', '1');
      |         set_param(gcb,'ulim','65535');
      |         set_param(gcb,'dlim','0');
      |         set_param(gcb,'unit','1 hex to decimal');
      |     case '0x2C'
      |         set_param(gcb, 'resol', '.01');
      |         set_param(gcb,'ulim','655.35');
      |         set_param(gcb,'dlim','0');
      |         set_param(gcb,'unit','0.01 g/cyl per bit');
      |     case '0x2D'
      |         set_param(gcb, 'resol', '.01');
      |         set_param(gcb,'ulim','655.35');
      |         set_param(gcb,'dlim','0');
      |         set_param(gcb,'unit','0.01 mg/stroke');
      |     case '0x2E'
      |         set_param(gcb, 'resol', '1');
      |         set_param(gcb,'ulim','1');
      |         set_param(gcb,'dlim','0');
      |         set_param(gcb,'unit','state encoded,');
      |     case '0x2F'
      |         set_param(gcb, 'resol', '.01');
      |         set_param(gcb,'ulim','655.35');
      |         set_param(gcb,'dlim','0');
      |         set_param(gcb,'unit','0.01 % per bit');
      |     case '0x30'
      |         set_param(gcb, 'resol', '0.001526');
      |         set_param(gcb,'ulim','100.00641');
      |         set_param(gcb,'dlim','0');
      |         set_param(gcb,'unit','0.001526 % per bit');
      |     case '0x31'
      |         set_param(gcb, 'resol', '.001');
      |         set_param(gcb,'ulim','65.535');
      |         set_param(gcb,'dlim','0');
      |         set_param(gcb,'unit','0.001 L per bit');
      |     case '0x32'
      |         set_param(gcb, 'resol', '0.00003051757813');
      |         set_param(gcb,'ulim','1.99996948274955');
      |         set_param(gcb,'dlim','0');
      |         set_param(gcb,'unit','0.000030517578 inch per bit');
      |     case '0x33'
      |         set_param(gcb, 'resol', '0.000244140625');
      |         set_param(gcb,'ulim','15.999755859375');
      |         set_param(gcb,'dlim','0');
      |         set_param(gcb,'unit','0.00024414 per bit');
      |     case '0x34'
      |         set_param(gcb, 'resol', '1');
      |         set_param(gcb,'ulim','65535');
      |         set_param(gcb,'dlim','0');
      |         set_param(gcb,'unit','1 minute per bit');
      |     case '0x35'
      |         set_param(gcb, 'resol', '10');
      |         set_param(gcb,'ulim','655350');
      |         set_param(gcb,'dlim','0');
      |         set_param(gcb,'unit','10 ms per bit');
      |     case '0x36'
      |         set_param(gcb, 'resol', '0.01');
      |         set_param(gcb,'ulim','655.35');
      |         set_param(gcb,'dlim','0');
      |         set_param(gcb,'unit','0.01 g per bit');
      |     case '0x37'
      |         set_param(gcb, 'resol', '0.1');
      |         set_param(gcb,'ulim','6553.5');
      |         set_param(gcb,'dlim','0');
      |         set_param(gcb,'unit','0.1 g per bit');
      |     case '0x38'
      |         set_param(gcb, 'resol', '1');
      |         set_param(gcb,'ulim','65535');
      |         set_param(gcb,'dlim','0');
      |         set_param(gcb,'unit','1 g per bit');
      |     case '0x39'
      |         set_param(gcb, 'resol', '.01');
      |         set_param(gcb,'ulim','655.35');
      |         set_param(gcb,'dlim','0');
      |         set_param(gcb,'unit','0.01 % per bit');
      |     case '0x3A'
      |         set_param(gcb, 'resol', '0.001');
      |         set_param(gcb,'ulim','65.535');
      |         set_param(gcb,'dlim','0');
      |         set_param(gcb,'unit','0.001 g per bit');
      |     case '0x3B'
      |         set_param(gcb, 'resol', '0.0001');
      |         set_param(gcb,'ulim','6.5535');
      |         set_param(gcb,'dlim','0');
      |         set_param(gcb,'unit','0.0001 g per bit');
      |     case '0x3C'
      |         set_param(gcb, 'resol', '0.1');
      |         set_param(gcb,'ulim','6553.5');
      |         set_param(gcb,'dlim','0');
      |         set_param(gcb,'unit','0.1 ms per bit');
      |     case '0x3D'
      |         set_param(gcb, 'resol', '.01');
      |         set_param(gcb,'ulim','655.35');
      |         set_param(gcb,'dlim','0');
      |         set_param(gcb,'unit','0.01 A per bit');
      |     case '0x3E'
      |         set_param(gcb, 'resol', '0.00006103516');
      |         set_param(gcb,'ulim','3.9999392106');
      |         set_param(gcb,'dlim','0');
      |         set_param(gcb,'unit','0.00006103516  mm2 per bit');
      |     case '0x3F'
      |         set_param(gcb, 'resol', '0.01');
      |         set_param(gcb,'ulim','655.35');
      |         set_param(gcb,'dlim','0');
      |         set_param(gcb,'unit','0.01 L per bit');
      |     case '0x40'
      |         set_param(gcb, 'resol', '1');
      |         set_param(gcb,'ulim','65535');
      |         set_param(gcb,'dlim','0');
      |         set_param(gcb,'unit','1 ppm per bit');
      |     case '0x41'
      |         set_param(gcb, 'resol', '0.01');
      |         set_param(gcb,'ulim','655.35');
      |         set_param(gcb,'dlim','0');
      |         set_param(gcb,'unit','0.01 mA per bit');
      |     case '0x42'
      |         set_param(gcb, 'resol', '0.1');
      |         set_param(gcb,'ulim','6553.5');
      |         set_param(gcb,'dlim','0');
      |         set_param(gcb,'unit','0.1 kJ per bit');
      |     case '0x43'
      |         set_param(gcb, 'resol', '0.000244140625');
      |         set_param(gcb,'ulim','15.999755859375');
      |         set_param(gcb,'dlim','0');
      |         set_param(gcb,'unit','0.00024414 g/kWh per bit');
      |     case '0x44'
      |         set_param(gcb, 'resol', '1');
      |         set_param(gcb,'ulim','65535');
      |         set_param(gcb,'dlim','0');
      |         set_param(gcb,'unit','1  S per cm per bit');
      |     case '0x81'
      |         set_param(gcb, 'resol', '1');
      |         set_param(gcb,'ulim','32767');
      |         set_param(gcb,'dlim','-32768');
      |         set_param(gcb,'unit','1 per bit');
      |     case '0x82'
      |         set_param(gcb, 'resol', '0.1');
      |         set_param(gcb,'ulim','3276.7');
      |         set_param(gcb,'dlim','-3276.8');
      |         set_param(gcb,'unit','0.1 per bit');
      |     case '0x83'
      |         set_param(gcb, 'resol', '0.01');
      |         set_param(gcb,'ulim','327.67');
      |         set_param(gcb,'dlim','-327.68');
      |         set_param(gcb,'unit','0.01 per bit');
      |     case '0x84'
      |         set_param(gcb, 'resol', '0.001');
      |         set_param(gcb,'ulim','32.767');
      |         set_param(gcb,'dlim','-32.768');
      |         set_param(gcb,'unit','0.001 per bit');
      |     case '0x85'
      |         set_param(gcb, 'resol', '0.000030517578');
      |         set_param(gcb,'ulim','0.999969478326');
      |         set_param(gcb,'dlim','-0.999999995904');
      |         set_param(gcb,'unit','0.000030517578 per bit');
      |     case '0x86'
      |         set_param(gcb, 'resol', '0.000305');
      |         set_param(gcb,'ulim','9.993935');
      |         set_param(gcb,'dlim','-9.99424');
      |         set_param(gcb,'unit','0.000305 per bit');
      |     case '0x87'
      |         set_param(gcb, 'resol', '1');
      |         set_param(gcb,'ulim','32767');
      |         set_param(gcb,'dlim','-32768');
      |         set_param(gcb,'unit','1 ppm per bit');
      |     case '0x8A'
      |         set_param(gcb, 'resol', '0.1220703125');
      |         set_param(gcb,'ulim','3999.8779296875');
      |         set_param(gcb,'dlim','-4000');
      |         set_param(gcb,'unit','0.1220703125 mV per bit');
      |     case '0x8B'
      |         set_param(gcb, 'resol', '0.001');
      |         set_param(gcb,'ulim','32.767');
      |         set_param(gcb,'dlim','-32.768');
      |         set_param(gcb,'unit','0.001 V per bit');
      |     case '0x8C'
      |         set_param(gcb, 'resol', '0.01');
      |         set_param(gcb,'ulim','327.67');
      |         set_param(gcb,'dlim','-327.68');
      |         set_param(gcb,'unit','0.01 V per bit');
      |     case '0x8D'
      |         set_param(gcb, 'resol', '0.00390625');
      |         set_param(gcb,'ulim','127.99609375');
      |         set_param(gcb,'dlim','-128');
      |         set_param(gcb,'unit','0.00390625 mA per bit');
      |     case '0x8E'
      |         set_param(gcb, 'resol', '0.001');
      |         set_param(gcb,'ulim','32.767');
      |         set_param(gcb,'dlim','-32.768');
      |         set_param(gcb,'unit','0.001 mA per bit');
      |     case '0x8F'
      |         set_param(gcb, 'resol', '1');
      |         set_param(gcb,'ulim','32767');
      |         set_param(gcb,'dlim','-32768');
      |         set_param(gcb,'unit','1 ms per bit');
      |     case '0x90'
      |         set_param(gcb, 'resol', '1');
      |         set_param(gcb,'ulim','32767');
      |         set_param(gcb,'dlim','-32768');
      |         set_param(gcb,'unit','1 ms per bit');
      |     case '0x91'
      |         set_param(gcb, 'resol', '0.1');
      |         set_param(gcb,'ulim','3276.7');
      |         set_param(gcb,'dlim','-3276.8');
      |         set_param(gcb,'unit','0.1 s per bit');
      |     case '0x92'
      |         set_param(gcb, 'resol', '0.1');
      |         set_param(gcb,'ulim','3276.7');
      |         set_param(gcb,'dlim','-3276.8');
      |         set_param(gcb,'unit','0.1 Nm per bit');
      |     case '0x96'
      |         set_param(gcb, 'resol', '0.1');
      |         set_param(gcb,'ulim','3276.7');
      |         set_param(gcb,'dlim','-3276.8');
      |         set_param(gcb,'unit','0.1 oC per bit');
      |     case '0x97'
      |         set_param(gcb, 'resol', '0.01');
      |         set_param(gcb,'ulim','327.67');
      |         set_param(gcb,'dlim','-327.68');
      |         set_param(gcb,'unit','0.01 oC/s per bit');
      |     case '0x98'
      |         set_param(gcb, 'resol', '1');
      |         set_param(gcb,'ulim','32767');
      |         set_param(gcb,'dlim','-32768');
      |         set_param(gcb,'unit','1 mg/stroke per bit');
      |     case '0x99'
      |         set_param(gcb, 'resol', '0.1');
      |         set_param(gcb,'ulim','3276.7');
      |         set_param(gcb,'dlim','-3276.8');
      |         set_param(gcb,'unit','0.1 kPa per bit');
      |     case '0x9C'
      |         set_param(gcb, 'resol', '0.01');
      |         set_param(gcb,'ulim','327.67');
      |         set_param(gcb,'dlim','-327.68');
      |         set_param(gcb,'unit','0.01 o per bit');
      |     case '0x9D'
      |         set_param(gcb, 'resol', '0.5');
      |         set_param(gcb,'ulim','16383.5');
      |         set_param(gcb,'dlim','-16384');
      |         set_param(gcb,'unit','0.5 o per bit');
      |     case '0xA8'
      |         set_param(gcb, 'resol', '1');
      |         set_param(gcb,'ulim','32767');
      |         set_param(gcb,'dlim','-32768');
      |         set_param(gcb,'unit','1 g/s per bit');
      |     case '0xA9'
      |         set_param(gcb, 'resol', '0.25');
      |         set_param(gcb,'ulim','8191.75');
      |         set_param(gcb,'dlim','-8192');
      |         set_param(gcb,'unit','0.25 Pa/s per bit');
      |     case '0xAD'
      |         set_param(gcb, 'resol', '0.01');
      |         set_param(gcb,'ulim','327.67');
      |         set_param(gcb,'dlim','-327.68');
      |         set_param(gcb,'unit','0.01 mg/stroke per bit');
      |     case '0xAE'
      |         set_param(gcb, 'resol', '0.1');
      |         set_param(gcb,'ulim','3276.7');
      |         set_param(gcb,'dlim','-3276.8');
      |         set_param(gcb,'unit','0.1 mg/stroke per bit');
      |     case '0xAF'
      |         set_param(gcb, 'resol', '0.01');
      |         set_param(gcb,'ulim','327.67');
      |         set_param(gcb,'dlim','-327.68');
      |         set_param(gcb,'unit','0.01 % per bit');
      |     case '0xB0'
      |         set_param(gcb, 'resol', '0.003052');
      |         set_param(gcb,'ulim','100.004884');
      |         set_param(gcb,'dlim','-100.007936');
      |         set_param(gcb,'unit','0.003052 % per bit');
      |     case '0xB1'
      |         set_param(gcb, 'resol', '2');
      |         set_param(gcb,'ulim','65534');
      |         set_param(gcb,'dlim','-65536');
      |         set_param(gcb,'unit','2mV/s per bit');
      |     case '0xFA'
      |         set_param(gcb, 'resol', '20');
      |         set_param(gcb,'ulim','655340');
      |         set_param(gcb,'dlim','-655360');
      |         set_param(gcb,'unit','20 kPa per bit');
      |     case '0xFB'
      |         set_param(gcb, 'resol', '10');
      |         set_param(gcb,'ulim','327670');
      |         set_param(gcb,'dlim','-327680');
      |         set_param(gcb,'unit','10 kPa per bit');
      |     case '0xFC'
      |         set_param(gcb, 'resol', '0.01');
      |         set_param(gcb,'ulim','327.67');
      |         set_param(gcb,'dlim','-327.68');
      |         set_param(gcb,'unit','0.01 kPa per bit');
      |     case '0xFD'
      |         set_param(gcb, 'resol', '0.001');
      |         set_param(gcb,'ulim','32.767');
      |         set_param(gcb,'dlim','-32.768');
      |         set_param(gcb,'unit','0.001 kPa per bit');
      |     case '0xFE'
      |         set_param(gcb, 'resol', '0.25');
      |         set_param(gcb,'ulim','8191.75');
      |         set_param(gcb,'dlim','-8192');
      |         set_param(gcb,'unit','0.25 Pa per bit');
      | end
      | clear contype_case;
      mask Display:
      | blk_handle = gcbh;
      | try
      |     set(blk_handle,'MaskIconOpaque','transparent');
      | catch
      |     set(blk_handle,'MaskIconOpaque','off');
      | end
      | 
      | if strcmpi(Specificchoix,'on')
      |     dgn_mask = [char(EventId) '\n \n Dimension : ' Dim_num '\n Conversion : ' conv_type '\n \n Resolution & Unit :' unit '\n Upper Limit :' ulim '\n Lower Limit :' dlim ];
      |     set(blk_handle,'AttributesFormatString','%<MaskType>\nDTR Id : = %<EventId>\nSpecific case used only for Nissan cases = %<Specificchoix>\nDimension : = %<Dim_num>\nConversion Type = %<conv_type>\nResolution and Unit : = %<unit>\nLower Limit : = %<dlim>\nUpper Limit : = %<ulim>');
      | else
      |     dgn_mask = [char(EventId) '\n \n Conversion : ' conv_type '\n \n Resolution & Unit :' unit '\n Upper Limit :' ulim '\n Lower Limit :' dlim ];
      |     set(blk_handle,'AttributesFormatString','%<MaskType>\nDTR Id : = %<EventId>\nSpecific case used only for Nissan cases = %<Specificchoix>\nConversion Type = %<conv_type>\nResolution and Unit : = %<unit>\nLower Limit : = %<dlim>\nUpper Limit : = %<ulim>');
      | end
      | 
      | 
      | disp(dgn_mask);
      | plot([5,5,5])
      | plot([6,6,6])
  AEMS_DEM_SET_ENBL_COND : Subsystem  Tag=[LIB]  mask(AEMS_DEM_SET_ENBL_COND){EnCondId=Dem_EnableConditionId_XXX, Specificchoix=off, Dim_num=1}
      mask prompts: EnCondId "Enable Condition Id"; Specificchoix "Specific case used only for Nissan cases"; Dim_num "Dimension :"
      mask help:
      | [SWS_Dem_00201]
      |
      | Sets an enable condition.
      mask init:
      | % EnCondId = ['Dem_EnableConditionId_' DiagName];
      | EnCondId = get_param(gcb,'EnCondId');
      | eval([char(EnCondId) ' = 0;']);
      | 
      | lib_path = gcb;
      | child_lib = find_system(lib_path,'LookUnderMasks','all','FollowLinks','on','Name','DEM_SET_ENBL_COND_D');
      | 
      | if strcmpi(Specificchoix,'off')
      |     Dim_num='1';
      | end
      | 
      | switch Dim_num
      |     case '1'
      |         blk_rep = 'AEMS_DEM_SET_ENBL_COND_1D';
      |     case '2'
      |         blk_rep = 'AEMS_DEM_SET_ENBL_COND_2D';
      |     case '8'
      |         blk_rep = 'AEMS_DEM_SET_ENBL_COND_8D';
      | end
      | 
      | if ismember(get_param(child_lib,'MaskType'),{blk_rep})
      | else
      |     replace_block(lib_path,'FollowLinks','on','Name','DEM_SET_ENBL_COND_D',['AEMS_Standard_Library/SUB/',blk_rep],'noprompt');
      | end
      | 
      | % set_param([child_lib{:}],'DiagName',char(DiagName));
      | set_param([child_lib{:}],'EnCondId',char(EnCondId));
      settings: AttributesFormatString=%<MaskType>\nEnable Condition Id = %<EnCondId>\nSpecific case used only for Nissan cases = %<Specificchoix>
      mask Callback EnCondId: % set_param(gcb,'EnCondId',['Dem_EnableConditionId_' get_param(gcb,'DiagName')]);
      mask Callback Specificchoix:
      | maskobj = Simulink.Mask.get(gcbh);
      | maskobj_param = maskobj.Parameters;
      | if strcmp(get(gcbh,'Specificchoix'),'on')
      |     maskobj_param(3).Visible = 'on';
      |     maskobj_param(3).Enabled = 'on';
      | else
      |     maskobj_param(3).Visible = 'off';
      |     maskobj_param(3).Enabled = 'off';
      | end
      | clear maskobj_param;
      | clear maskobj;
      mask TypeOptions Dim_num: 1 | 2 | 8
      mask Display:
      | port_label('input',1,'conditionfulfilled');
      | 
      | if strcmpi(Specificchoix,'on')
      |     dgn_mask = [char(EnCondId) '\n Dimension : ' Dim_num];
      |     set(gcbh,'AttributesFormatString','%<MaskType>\nEnable Condition Id = %<EnCondId>\nSpecific case used only for Nissan cases = %<Specificchoix>\nDimension : = %<Dim_num>');
      | else
      |     dgn_mask = char(EnCondId);
      |     set(gcbh,'AttributesFormatString','%<MaskType>\nEnable Condition Id = %<EnCondId>\nSpecific case used only for Nissan cases = %<Specificchoix>');
      | end
      | 
      | disp(dgn_mask);
      | 
      | plot([5,5,5])
      | plot([6,6,6])
  AEMS_DEM_SET_EVENT_AVL : Subsystem  Tag=[LIB]  mask(AEMS_DEM_SET_EVENT_AVL){EventID=Dem_EventId, DiagROMFLAG=Diag_ROMFLAG, Specificchoix=off, Dim_num=-	(1 dimension), immediate=}
      mask prompts: EventID "Identification of an event :"; DiagROMFLAG "Diagnosis ROMFLAG :"; Specificchoix "Specific case used only for Nissan cases"; Dim_num "index immediate :"
      mask help:
      | [Set Event Available]
      | - Set the available status of a specific Event.
      | - "Set Event Available" must be placed in diagnosis models to send
      |  enable/disable diagnosis request for DEM.
      | - "Set Event Available" includes Diagnosis ROM flag inside of library.
      | - "Set Event Available" outputs the DGNSW signal.
      | - Refer the AUTOSAR Dem_SetEventAvailable [SWS_Dem_01080]
      |
      | -OUTPUTS-
      | - DGNSW outputs are used to enable/disable diagnosis in models.
      |
      | -PARAMETERS-
      | EventId: Identification of an event
      | Diagnosis ROMFLAG: Diagnosis ROMFLAG
      |
      | When specific case used only for Nissan cases is checked:
      | index immediate: If diagnosis has more than 2 dimension, select
      | "index immediate" and add iXXX immediate in Dataobject file(_ROM)
      mask init:
      | % EventId = ['Dem_EventId_' DiagName];
      | % DiagROMFLAG = ['mf' DiagName];
      | eval([char(EventID) '= 0;'])%EventId is defined only in the library
      | lib_path = gcb;
      | if strcmpi(Specificchoix,'off')
      |    Dim_num='(1 dimension )';
      | end
      | %Specify child
      | child_lib = find_system(lib_path,'LookUnderMasks','all','FollowLinks','on','Name','DEM_SET_EVENT_AVL_D');
      | 
      | %Change the library structure
      | if ismember('(1 dimension )',char(Dim_num))
      |     if ismember(get_param(child_lib,'MaskType'),{'AEMS_DEM_SET_EVENT_AVL_1D'})
      |     else
      |         replace_block(lib_path,'FollowLinks','on','Name','DEM_SET_EVENT_AVL_D','AEMS_Standard_Library/SUB/AEMS_DEM_SET_EVENT_AVL_1D','noprompt');
      |     end
      |     
      |     % Set immediate typefor parent block
      |     set_param(lib_path,'immediate','');
      |     
      | elseif ismember('iBANK',char(Dim_num))
      |     if ismember(get_param(child_lib,'MaskType'),{'AEMS_DEM_SET_EVENT_AVL_2D'})
      |     else
      |         replace_block(lib_path,'FollowLinks','on','Name','DEM_SET_EVENT_AVL_D','AEMS_Standard_Library/SUB/AEMS_DEM_SET_EVENT_AVL_2D','noprompt');
      |     end
      |     % Set immediate type (only 2 dimensions)
      |     set_param([child_lib{:}],'immediate','Cnx_bnk_nr_conf');
      |     % Set sample_time
      |     set_param([child_lib{:}],'sample_time','-1');
      |     % Set immediate typefor parent block
      |     set_param(lib_path,'immediate','Cnx_bnk_nr_conf');
      |     
      | elseif ismember('iTHROTTLE',char(Dim_num))
      |     if ismember(get_param(child_lib,'MaskType'),{'AEMS_DEM_SET_EVENT_AVL_2D'})
      |     else
      |         replace_block(lib_path,'FollowLinks','on','Name','DEM_SET_EVENT_AVL_D','AEMS_Standard_Library/SUB/AEMS_DEM_SET_EVENT_AVL_2D','noprompt');
      |     end
      |     % Set immediate type (only 2 dimensions)
      |     set_param([child_lib{:}],'immediate','Cnx_thr_nr_conf');
      |     % Set sample_time
      |     set_param([child_lib{:}],'sample_time','-1');
      |     % Set immediate typefor parent block
      |     set_param(lib_path,'immediate','Cnx_thr_nr_conf');
      |     
      | elseif ismember('iAIR_FLOW_METER',char(Dim_num))
      |     if ismember(get_param(child_lib,'MaskType'),{'AEMS_DEM_SET_EVENT_AVL_2D'})
      |     else
      |         replace_block(lib_path,'FollowLinks','on','Name','DEM_SET_EVENT_AVL_D','AEMS_Standard_Library/SUB/AEMS_DEM_SET_EVENT_AVL_2D','noprompt');
      |     end
      |     % Set immediate type (only 2 dimensions)
      |     set_param([child_lib{:}],'immediate','Cnx_inairflw_nr_conf');
      |     % Set sample_time
      |     set_param([child_lib{:}],'sample_time','-1');    
      |     % Set immediate typefor parent block
      |     set_param(lib_path,'immediate','Cnx_inairflw_nr_conf');
      |     
      | elseif ismember('iCYLNDER',char(Dim_num))
      |     if ismember(get_param(child_lib,'MaskType'),{'AEMS_DEM_SET_EVENT_AVL_8D'})
      |     else
      |         replace_block(lib_path,'FollowLinks','on','Name','DEM_SET_EVENT_AVL_D','AEMS_Standard_Library/SUB/AEMS_DEM_SET_EVENT_AVL_8D','noprompt');
      |     end
      |     % Set sample_time
      |     set_param([child_lib{:}],'sample_time','-1');
      |     % Set immediate typefor parent block
      |     set_param(lib_path,'immediate','Cnx_cyl_nr_conf');
      | 
      | elseif ismember('MISFIRE',char(Dim_num))
      |     if ismember(get_param(child_lib,'MaskType'),{'AEMS_DEM_SET_EVENT_AVL_9D'})
      |     else
      |         replace_block(lib_path,'FollowLinks','on','Name','DEM_SET_EVENT_AVL_D','AEMS_Standard_Library/SUB/AEMS_DEM_SET_EVENT_AVL_9D','noprompt');
      |     end
      |     % Set sample_time
      |     set_param([child_lib{:}],'sample_time','-1');
      |     % Set immediate typefor parent block
      |     set_param(lib_path,'immediate','Cnx_cyl_nr_conf');
      | end
      | 
      | 
      | %Set Diagnosis parameters
      | set_param([child_lib{:}],'EventId',char(EventID));
      | set_param([child_lib{:}],'DiagROMFLAG',char(DiagROMFLAG));
      settings: AttributesFormatString=%<MaskType>\nIdentification of an event : = %<EventID>\nDiagnosis ROMFLAG : = %<DiagROMFLAG>\nSpecific case used only for Nissan cases = %<Specificchoix>
      mask Help:
      | eval('path_lib=fileparts(which(''AEMS_Standard_Library''));');
      | mskblk=get_param(gcbh,'MaskType');
      | doc_path = [path_lib '\help\',mskblk,'.pdf'];
      | eval('open(doc_path)');
      mask Callback Specificchoix:
      | maskobj = Simulink.Mask.get(gcbh);
      | maskobj_param = maskobj.Parameters;
      | if strcmp(get(gcbh,'Specificchoix'),'on')
      |     maskobj_param(4).Visible = 'on';
      |     maskobj_param(4).Enabled = 'on';
      | else
      |     maskobj_param(4).Visible = 'off';
      |     maskobj_param(4).Enabled = 'off';
      | end
      | clear maskobj;
      | clear maskobj_param;
      mask TypeOptions Dim_num: -	(1 dimension) | iBANK	(2 dimensions) | iTHROTTLE	(2 dimensions) | iAIR_FLOW_METER (2 dimensions) | iCYLNDER	(8 dimensions) | MISFIRE	(9 dimensions)
      mask Display:
      | port_label('output',1,'dgnsw');
      | 
      | if strcmpi(Specificchoix,'on')
      |     dgn_mask = ['Identification of an event: ',char(EventID),'\n Diagnosis ROMFLAG: ',char(DiagROMFLAG),'\n index immediate : ',Dim_num];
      |     set_param(gcb,'AttributesFormatString','%<MaskType>\nIdentification of an event : = %<EventID>\nDiagnosis ROMFLAG : = %<DiagROMFLAG>\nSpecific case used only for Nissan cases = %<Specificchoix>\nindex immediate : = %<Dim_num>');
      | else
      |     dgn_mask = ['Identification of an event: ',char(EventID),'\n Diagnosis ROMFLAG: ',char(DiagROMFLAG),'\n'];
      |     set_param(gcb,'AttributesFormatString','%<MaskType>\nIdentification of an event : = %<EventID>\nDiagnosis ROMFLAG : = %<DiagROMFLAG>\nSpecific case used only for Nissan cases = %<Specificchoix>');
      | end
      | 
      | disp(dgn_mask);
      | plot([5,5,5])
      | plot([6,6,6])
  AEMS_DEM_SET_EVENT_DSBL : Subsystem  Tag=[LIB]  mask(AEMS_DEM_SET_EVENT_DSBL){EventId=Dem_EventId_XXX, Specificchoix=off, Dim_num=1}
      mask prompts: EventId "EventId :"; Specificchoix "Specific case used only for Nissan cases"; Dim_num "Dimension :"
      mask help:
      | Dem_SetEventDisabled [SWS_Dem_00312]
      | Service for reporting the event as disabled to the Dem for the PID 41
      | computation.
      |
      | Dimension: Select dimension corresponding to diagnosis dimension
      |
      | EventId: Automatically filled
      mask init:
      | % EventId = ['Dem_EventId_' DiagName];
      | EventId = get_param(gcb,'EventId');
      | eval([char(EventId) '= 0;'])
      | lib_path = gcb;
      | 
      | %Specify child
      | child_lib = find_system(lib_path,'LookUnderMasks','all','FollowLinks','on','Name','DEM_SET_EVENT_DSBL_D');
      | 
      | if strcmpi(Specificchoix,'off')
      |     Dim_num='1';
      | end
      | 
      | switch Dim_num
      |     case '1'
      |         blk_rep = 'AEMS_DEM_SET_EVENT_DSBL_1D';
      |     case '2'
      |         blk_rep = 'AEMS_DEM_SET_EVENT_DSBL_2D';
      |     case '8'
      |         blk_rep = 'AEMS_DEM_SET_EVENT_DSBL_8D';
      |     case '9'
      |         blk_rep = 'AEMS_DEM_SET_EVENT_DSBL_9D';
      | end
      | if ismember(get_param(child_lib,'MaskType'),{blk_rep})
      | else
      |     replace_block(lib_path,'FollowLinks','on','Name','DEM_SET_EVENT_DSBL_D',['AEMS_Standard_Library/SUB/',blk_rep],'noprompt');
      | end
      | 
      | %Set Diagnosis parameters
      | % set_param([child_lib{:}],'DiagName',char(DiagName));
      | set_param([child_lib{:}],'EventId',char(EventId));
      settings: AttributesFormatString=%<MaskType>\nEventId : = %<EventId>\nSpecific case used only for Nissan cases = %<Specificchoix>
      mask Help:
      | eval('path_lib=fileparts(which(''AEMS_Standard_Library''));');
      | doc_path = [path_lib '\help\AEMS_DEM_SET_EVENT_DSBL.pdf'];
      | eval('open(doc_path)')
      mask Callback Specificchoix:
      | maskobj = Simulink.Mask.get(gcbh);
      | maskobj_param = maskobj.Parameters;
      | if strcmp(get(gcbh,'Specificchoix'),'on')
      |     maskobj_param(3).Visible = 'on';
      |     maskobj_param(3).Enabled = 'on';
      | else
      |     maskobj_param(3).Visible = 'off';
      |     maskobj_param(3).Enabled = 'off';
      | end
      | clear maskobj_param;
      | clear maskobj;
      mask TypeOptions Dim_num: 1 | 2 | 8 | 9
      mask Display:
      | port_label('input',1,'set_flag');
      | 
      | if strcmpi(Specificchoix,'on')
      | dgn_mask = [EventId,'\nDimension : ',Dim_num];
      | set(gcbh,'AttributesFormatString','%<MaskType>\nEventId : = %<EventId>\nSpecific case used only for Nissan cases = %<Specificchoix>\nDimension : = %<Dim_num>');
      | else
      | dgn_mask = [EventId];
      | set(gcbh,'AttributesFormatString','%<MaskType>\nEventId : = %<EventId>\nSpecific case used only for Nissan cases = %<Specificchoix>');
      | end
      | 
      | disp(dgn_mask);
      | plot([5,5,5])
      | plot([6,6,6])
  AEMS_DEM_SET_EVENT_STS : Subsystem  Tag=[LIB]  mask(AEMS_DEM_SET_EVENT_STS){EventId=Dem_EventId_XXX, LibType=_DGNTRP, Specificchoix=off, Dim_num=1}
      mask prompts: EventId "EventId :"; LibType "DEM Library type :"; Specificchoix "Specific case used only for Nissan cases"; Dim_num "Dimension :"
      mask help:
      | [Set Event Status]
      | - Set the diagnosis event status reported by SW-Cs via RTE.
      | - "Set Event Status" must be placed in all diagnosis models including confirmation of diagnosis failure/no failure.
      | - Refer the AUTOSAR Dem_SetEventStatus [SWS_Dem_00183]
      |
      | DEM Library type:
      | Select type of diagnosis result
      | xxx_DGNTRP-- To confirm failure
      | xxx_DGNOK--- To confirm OK judgment
      |
      | Dimension: Select dimension corresponding to diagnosis dimension
      |
      | EventId: Diagnosis Event ID
      mask init:
      | % EventId = ['Dem_EventId_' DiagName];D
      | EventId = get_param(gcb,'EventId');
      | eval([char(EventId) '= 0;'])
      | lib_path = gcb;
      | 
      | %Specify child
      | child_lib = find_system(lib_path,'LookUnderMasks','all','FollowLinks','on','Name','AEMS_DEM_SET_EVENT_STS_D');
      | 
      | if strcmpi(Specificchoix,'off')
      |    Dim_num = '1';
      | end
      | 
      | switch Dim_num
      |     case '1'
      |         if ismember(get_param(child_lib,'MaskType'),{'AEMS_DEM_SET_EVENT_STS_1D'})
      |         else
      |             replace_block(lib_path,'FollowLinks','on','Name','AEMS_DEM_SET_EVENT_STS_D','AEMS_Standard_Library/SUB/AEMS_DEM_SET_EVENT_STS_1D','noprompt');
      |         end
      |     case '2'
      |         if ismember(get_param(child_lib,'MaskType'),{'AEMS_DEM_SET_EVENT_STS_2D'})
      |         else
      |             replace_block(lib_path,'FollowLinks','on','Name','AEMS_DEM_SET_EVENT_STS_D','AEMS_Standard_Library/SUB/AEMS_DEM_SET_EVENT_STS_2D','noprompt');
      |         end
      |     case '8'
      |         if ismember(get_param(child_lib,'MaskType'),{'AEMS_DEM_SET_EVENT_STS_8D'})
      |         else
      |             replace_block(lib_path,'FollowLinks','on','Name','AEMS_DEM_SET_EVENT_STS_D','AEMS_Standard_Library/SUB/AEMS_DEM_SET_EVENT_STS_8D','noprompt');
      |         end        
      |     case '9'
      |         if ismember(get_param(child_lib,'MaskType'),{'AEMS_DEM_SET_EVENT_STS_9D'})
      |         else
      |             replace_block(lib_path,'FollowLinks','on','Name','AEMS_DEM_SET_EVENT_STS_D','AEMS_Standard_Library/SUB/AEMS_DEM_SET_EVENT_STS_9D','noprompt');
      |         end
      | end
      | 
      | %Set Diagnosis parameters
      | % set_param([child_lib{:}],'DiagName',char(DiagName));
      | set_param([child_lib{:}],'EventId',char(EventId));
      | set_param([child_lib{:}],'LibType',char(LibType));
      settings: AttributesFormatString=%<MaskType>\nEventId : = %<EventId>\nDEM Library type : = %<LibType>\nSpecific case used only for Nissan cases := %<Specificchoix>
      mask Help:
      | eval('path_lib=fileparts(which(''AEMS_Standard_Library''));');
      | doc_path = [path_lib '\help\AEMS_DEM_SET_EVENT_STS.pdf'];
      | eval('open(doc_path)')
      mask Callback EventId: set_param(gcb,'EventId',get_param(gcb,'EventId'));
      mask TypeOptions LibType: _DGNTRP | _DGNOK
      mask Callback Specificchoix:
      | maskobj = Simulink.Mask.get(gcbh);
      | maskobj_old = maskobj.Parameters;
      | if strcmp(get(gcbh,'Specificchoix'),'on')
      |     maskobj_old(4).Visible = 'on';
      |     maskobj_old(4).Enabled = 'on';
      | else
      |     maskobj_old(4).Visible = 'off';
      |     maskobj_old(4).Enabled = 'off';
      | end
      | clear maskobj_old;
      | clear maskobj;
      mask TypeOptions Dim_num: 1 | 2 | 8 | 9
      mask Display:
      | dgn_mask = '';
      | 
      | switch LibType
      |     case '_DGNTRP'
      |         dgn_mask = [dgn_mask 'EventId: ' EventId '\nFailed: ' '_DGNTRP'];
      |     case '_DGNOK'
      |         dgn_mask = [dgn_mask 'EventId: ' EventId '\nPassed: ' '_DGNOK'];
      | end
      | 
      | if strcmpi(Specificchoix,'on')
      |     set_param(gcb,'AttributesFormatString','%<MaskType>\nEventId : = %<EventId>\nDEM Library type : = %<LibType>\nSpecific case used only for Nissan cases := %<Specificchoix>\nDimension : = %<Dim_num>');
      | else
      |     set_param(gcb,'AttributesFormatString','%<MaskType>\nEventId : = %<EventId>\nDEM Library type : = %<LibType>\nSpecific case used only for Nissan cases := %<Specificchoix>');
      | end
      | 
      | % switch Dim_num
      | %     case '1'
      | %         dgn_mask = [dgn_mask '\n (1 dimension)'];
      | %     case '2'
      | %         dgn_mask = [dgn_mask '\n (2 dimensions)'];
      | %     case '8'
      | %         dgn_mask = [dgn_mask '\n (8 dimensions)'];
      | % end
      | 
      | 
      | 
      | 
      | disp(dgn_mask);
      | plot([5,5,5])
      | plot([6,6,6])
  AEMS_DEM_SET_IUMPR_DCOND : Subsystem  Tag=[LIB]  mask(AEMS_DEM_SET_IUMPR_DCOND){ConditionId=DEM_IUMPR_GENERAL_DENOMINATOR}
      mask prompts: ConditionId "ConditionId :"
      mask help:
      | [Set IUMPR Den Condition]
      |
      | - Refer the AUTOSAR Dem_SetIUMPRDenCondition [SWS_Dem_00733]
      mask init:
      | lib_path = gcb;
      | condid_b = find_system(lib_path,'LookUnderMasks','all','FollowLinks','on','Name','ConditionId_Block');
      | 
      | switch ConditionId
      |     case 'DEM_IUMPR_GENERAL_DENOMINATOR'
      |         eval([char(ConditionId) ' = 1;']);
      |     case 'DEM_IUMPR_DEN_COND_COLDSTART'
      |         eval([char(ConditionId) ' = 2;']);
      |     case 'DEM_IUMPR_DEN_COND_EVAP'
      |         eval([char(ConditionId) ' = 3;']);
      |     case 'DEM_IUMPR_DEN_COND_500MI'
      |         eval([char(ConditionId) ' = 4;']);
      | end
      | 
      | set_param([condid_b{:}],'Value',char(ConditionId));
      settings: AttributesFormatString=%<MaskType>\nConditionId : = %<ConditionId>
      mask Help: Dem_SetIUMPRDenCondition [SWS_Dem_00733]
      mask TypeOptions ConditionId: DEM_IUMPR_GENERAL_DENOMINATOR | DEM_IUMPR_DEN_COND_COLDSTART | DEM_IUMPR_DEN_COND_EVAP | DEM_IUMPR_DEN_COND_500MI
      mask Display:
      | switch ConditionId
      |     case 'DEM_IUMPR_GENERAL_DENOMINATOR'
      |         dgn_mask = ['ConditionId : 0x01 \n' char(ConditionId)];
      |     case 'DEM_IUMPR_DEN_COND_COLDSTART'
      |         dgn_mask = ['ConditionId : 0x02 \n' char(ConditionId)];
      |     case 'DEM_IUMPR_DEN_COND_EVAP'
      |         dgn_mask = ['ConditionId : 0x03 \n' char(ConditionId)];
      |     case 'DEM_IUMPR_DEN_COND_500MI'
      |         dgn_mask = ['ConditionId : 0x04 \n' char(ConditionId)];
      | end
      | 
      | port_label('input',1,'condition_status');
      | port_label('input',2,'set_flag');
      | 
      | 
      | disp(dgn_mask);
      | plot([5,5,5])
      | plot([6,6,6])
  AEMS_DEM_SET_OPCYC_STE : Subsystem  Tag=[LIB]  mask(AEMS_DEM_SET_OPCYC_STE){OperationCycleId=DEM_OPCYC_IGNITION}
      mask prompts: OperationCycleId "OperationCycleId :"
      mask help:
      | [Set Operation Cycle State]
      | - Refer the AUTOSAR Dem_SetOperationCycleState [SWS_Dem_00194]
      mask init:
      | eval([char(OperationCycleId) '= 0;']);
      | 
      | lib_path = gcb;
      | opcycid_b = find_system(lib_path,'LookUnderMasks','all','FollowLinks','on','Name','OperationCycleId_Block');
      | set_param([opcycid_b{:}],'Value',char(OperationCycleId));
      settings: AttributesFormatString=%<MaskType>\nOperationCycleId : = %<OperationCycleId>
      mask Help:
      | Dem_SetOperationCycleState [SWS_Dem_00194]
      | Sets an operation cycle state.
      | This API can only be used through the RTE and therefore no declaration is exported via Dem.h.
      | The interface has an asynchronous behavior to avoid exceeding of typical timing requirements on APIs if a large number of events has to be processed and during the re-initializations of the related monitors.
      | The asynchronous acknowledgements are the related InitMonitorForEvent callbacks.
      mask TypeOptions OperationCycleId: DEM_OPCYC_IGNITION | DEM_OPCYC_OBD_DCY | DEM_OPCYC_WARMUP
      mask Display:
      | dgn_mask = ['OperationCycleId : \n' OperationCycleId];
      | disp(dgn_mask);
      | 
      | port_label('input',1,'cycle_state');
      | port_label('input',2,'set_flag');
      | 
      | plot([5,5,5])
      | plot([6,6,6])
  AEMS_DEM_SET_PFC_CYC_QUALD : Subsystem  Tag=[LIB]  mask(AEMS_DEM_SET_PFC_CYC_QUALD){}
      mask help:
      | [Set Pfc Cycle Qualified]
      | Marks the current OBD driving cycle as having met the criteria for the PFC cycle.
      | API is needed in OBD-relevant ECUs only.
      | - Refer the AUTOSAR Dem_SetPfcCycleQualified [SWS_Dem_00739]
      settings: AttributesFormatString=%<MaskType>
      mask Help:
      | Dem_SetPfcCycleQualified [SWS_Dem_00739]
      | Marks the current OBD driving cycle as having met the criteria for the PFC cycle.
      | API is needed in OBD-relevant ECUs only.
      mask Display:
      | disp('Dem_SetPfcCycleQualified \n\n');
      | 
      | port_label('input',1,'set_flag');
      | 
      | plot([5,5,5])
      | plot([6,6,6])
  AEMS_DEM_SET_STORAGE_COND : Subsystem  Tag=[LIB]  mask(AEMS_DEM_SET_STORAGE_COND){StorageCondId=Dem_StorageConditionId_XXX, Specificchoix=off, Dim_num=1}
      mask prompts: StorageCondId "Storage Condition Id"; Specificchoix "Specific case used only for Nissan cases"; Dim_num "Dimension :"
      mask help:
      | [SWS_Dem_00556]
      |
      | Sets  storage condition.
      mask init:
      | % EnCondId = ['Dem_EnableConditionId_' DiagName];
      | StorageCondId = get_param(gcb,'StorageCondId');
      | eval([char(StorageCondId) ' = 0;']);
      | 
      | lib_path = gcb;
      | child_lib = find_system(lib_path,'LookUnderMasks','all','FollowLinks','on','Name','DEM_SET_STORAGE_COND_D');
      | 
      | if strcmpi(Specificchoix,'off')
      |     Dim_num='1';
      | end
      | 
      | switch Dim_num
      |     case '1'
      |         blk_rep = 'AEMS_DEM_SET_STORAGE_COND_1D';
      |     case '2'
      |         blk_rep = 'AEMS_DEM_SET_STORAGE_COND_2D';
      |     case '8'
      |         blk_rep = 'AEMS_DEM_SET_STORAGE_COND_8D';
      | end
      | 
      | if ismember(get_param(child_lib,'MaskType'),{blk_rep})
      | else
      |     replace_block(lib_path,'FollowLinks','on','Name','DEM_SET_STORAGE_COND_D',['AEMS_Standard_Library/SUB/',blk_rep],'noprompt');
      | end
      | 
      | % set_param([child_lib{:}],'DiagName',char(DiagName));
      | set_param([child_lib{:}],'StorageCondId',char(StorageCondId));
      settings: AttributesFormatString=%<MaskType>\nStorage Condition Id = %<StorageCondId>\nSpecific case used only for Nissan cases = %<Specificchoix>
      mask Callback Specificchoix:
      | maskobj = Simulink.Mask.get(gcbh);
      | maskobj_param = maskobj.Parameters;
      | if strcmp(get(gcbh,'Specificchoix'),'on')
      |     maskobj_param(3).Visible = 'on';
      |     maskobj_param(3).Enabled = 'on';
      | else
      |     maskobj_param(3).Visible = 'off';
      |     maskobj_param(3).Enabled = 'off';
      | end
      | clear maskobj_param;
      | clear maskobj;
      mask TypeOptions Dim_num: 1 | 2 | 8
      mask Display:
      | port_label('input',1,'conditionfulfilled');
      | 
      | if strcmpi(Specificchoix,'on')
      |     dgn_mask = [char(StorageCondId) '\n Dimension : ' Dim_num];
      |     set(gcbh,'AttributesFormatString','%<MaskType>\nStorage Condition Id = %<StorageCondId>\nSpecific case used only for Nissan cases = %<Specificchoix>\nDimension : = %<Dim_num>');
      | else
      |     dgn_mask = char(StorageCondId);
      |     set(gcbh,'AttributesFormatString','%<MaskType>\nStorage Condition Id = %<StorageCondId>\nSpecific case used only for Nissan cases = %<Specificchoix>');
      | end
      | 
      | disp(dgn_mask);
      | 
      | plot([5,5,5])
      | plot([6,6,6])
  AEMS_DEM_TIME_BASED_DEBOUNCE : Subsystem  Tag=[LIB]  Description=This subsystem is interface for self diagnosis standard calculated from similar condition and NG judgment.  mask(AEMS_DEM_TIME_BASED_DEBOUNCE){eventid=Dem_EventId_Device_Faulttype, Specificchoix=off, Dim_num=1, DemDebounceBehavior1=DEM_DEBOUNCE_FREEZE (0), DemDebounceBehavior2=DEM_DEBOUNCE_FREEZE (0), DemDebounceBehavior3=DEM_DEBOUNCE_FREEZE (0), DemDebounceBehavior4=DEM_DEBOUNCE_RESET (1), DemDebounceBehavior5=DEM_DEBOUNCE_RESET (1), DemDebounceBehavior6=DEM_DEBOUNCE_RESET (1), DemDebounceBehavior7=DEM_DEBOUNCE_FREEZE (0), DemDebounceBehavior8=DEM_DEBOUNCE_FREEZE (0), DemDebounceTimeFailedThreshold=Cxx_dem_fail_thd_Device_Faulttype, DemDebounceTimePassedThreshold=Cxx_dem_pass_thd_Device_Faulttype, DemTimeBypassFailure=Cbx_dem_byp_fail_Device_Faulttype, sampletime=0.01, ToDataStoreMemory=on}
      mask prompts: eventid "Identifier of a diagnostic event (EventId)"; Specificchoix "Specific case used only for Nissan cases"; Dim_num "Time_Based_Debounce_Dimention"; DemDebounceBehavior1 "Dem Debounce Behavior 1"; DemDebounceBehavior2 "Dem Debounce Behavior 2"; DemDebounceBehavior3 "Dem Debounce Behavior 3"; DemDebounceBehavior4 "Dem Debounce Behavior 4"; DemDebounceBehavior5 "Dem Debounce Behavior 5"; DemDebounceBehavior6 "Dem Debounce Behavior 6"; DemDebounceBehavior7 "Dem Debounce Behavior 7"; DemDebounceBehavior8 "Dem Debounce Behavior 8"; DemDebounceTimeFailedThreshold "Debounce Time Failed Threshold"; DemDebounceTimePassedThreshold "Debounce Time Passed Threshold"; DemTimeBypassFailure "Dem Debounce Time Bypass Failure"; sampletime "Sample Time"; ToDataStoreMemory "Write Output To Data Store Memory"
      mask help:
      | It  transmit the status Failed or Passed to the DEM. Accordingly,
      | some bits of the UDS DTC status byte changes synchronously or
      | asynchronously according to the configuration.
      |
      | -INPUTS-
      | conditionfulfilled: specifies whether the storage condition assigned to the StorageConditionId is fulfilled
      | prefailed: Monitor reports nonqualified test result pre-failed
      | prepassed: Monitor reports nonqualified test result pre-passed
      | ClearDataRequest:Clears the Data Request value
      | reseteventdebounce: Freeze or reset the internal debounce timer.
      |
      | -OUTPUTS-
      | debouncevalue_for_failed: Value of debounce when an event failed
      | debouncevalue_for_passed: Value of debounce when an event passed
      | failed: Diagnostic monitor reports an event failed
      | passed: Diagnostic monitor reports an event passed
      |
      | -PARAMETERS-
      | EventId: Internal identifier of a diagnostic event. 0 is not a valid value.
      | Debounce Behavior: The event debounce counter will be frozen or reset
      | (0 for FREEZE and 1 for RESET)
      | Debounce Time Failed Threshold: Defines the time out duration for
      | "Event Failed" qualification.
      | Debounce Time Passed Threshold: Defines the time out duration for
      | "Event Passed" qualification.
      mask init:
      | lib_path = gcb;
      | Current_Child_Lib_Path = find_system(lib_path,'LookUnderMasks','all','FollowLinks','on','Name','AEMS_DEM_TIME_BASED_DEBOUNCE_D');
      | Attribute_Format_String_Part1 = '%<MaskType>\n EventId : %<eventid> \n Specific case used only for Nissan cases = %<Specificchoix> ';
      | Attribute_Format_String_Part2 = '';
      | if strcmpi(Specificchoix,'off')
      |     Dim_num = '1';
      | else
      |     Attribute_Format_String_Part2 = '\n Time_Based_Debounce_Dimention = %<Dim_num> ';
      | end
      | dim_block = ['AEMS_DEM_TIME_BASED_DEBOUNCE_' Dim_num 'D'];
      | 
      | rep_block = ['AEMS_Standard_Library/SUB/',dim_block];
      | if ismember(get_param(Current_Child_Lib_Path,'MaskType'),{dim_block})
      | else
      |     replace_block(lib_path,'FollowLinks','on','Name','AEMS_DEM_TIME_BASED_DEBOUNCE_D',rep_block,'noprompt');
      | end
      | 
      | Attribute_Format_String_Part3='';
      | for i=1:str2num(Dim_num)
      |     Attribute_Format_String_Part3=[Attribute_Format_String_Part3,'\n Dem Debounce Behavior ',num2str(i),' = %<DemDebounceBehavior',num2str(i),'>'];
      |     set_param([Current_Child_Lib_Path{:}],['DemDebounceBehavior',num2str(i)],get_param(lib_path,['DemDebounceBehavior',num2str(i)]));
      | end
      | 
      | DemDebounceTimeFailedThreshold_tmp = get_param(lib_path,'DemDebounceTimeFailedThreshold');
      | DemDebounceTimePassedThreshold_tmp = get_param(lib_path,'DemDebounceTimePassedThreshold');
      | DemTimeBypassFailure_tmp = get_param(lib_path,'DemTimeBypassFailure');
      | sampletime_tmp = get_param(lib_path,'sampletime');
      | 
      | set_param([Current_Child_Lib_Path{:}],'eventid',eventid);
      | set_param([Current_Child_Lib_Path{:}],'DemDebounceTimeFailedThreshold',DemDebounceTimeFailedThreshold_tmp);
      | set_param([Current_Child_Lib_Path{:}],'DemDebounceTimePassedThreshold',DemDebounceTimePassedThreshold_tmp);
      | set_param([Current_Child_Lib_Path{:}],'DemTimeBypassFailure',DemTimeBypassFailure_tmp);
      | set_param([Current_Child_Lib_Path{:}],'Sample_Time',sampletime_tmp);
      | 
      | %If To DataStoreMemory is enabled...
      | if strcmpi(ToDataStoreMemory,'on')&& isempty(find_system(lib_path,'LookUnderMasks','all','FollowLinks','on','Name','AEMS_SRFLIPFLOP'))
      |     add_block('AEMS_Standard_Library/FLAG/AEMS_SRFLIPFLOP',[lib_path,'/AEMS_SRFLIPFLOP'],'Position',[930 254 1015 376]);
      |     add_block('simulink/Signal Attributes/Data Type Conversion',[lib_path,'/Data Type Conversion'],'Position',[1060 303 1115 327],'ShowName','off')
      |     add_block('simulink/Signal Routing/Data Store Write',[lib_path,'/Data Store Write'],'Position',[1160 302 1385 328],'ShowName','off');
      |     add_line(lib_path,'AEMS_DEM_TIME_BASED_DEBOUNCE_D/3','AEMS_SRFLIPFLOP/1','AutoRouting','on');
      |     add_line(lib_path,'AEMS_DEM_TIME_BASED_DEBOUNCE_D/4','AEMS_SRFLIPFLOP/2','AutoRouting','on');
      |     add_line(lib_path,'AEMS_SRFLIPFLOP/1','Data Type Conversion/1');
      |     add_line(lib_path,'Data Type Conversion/1','Data Store Write/1');
      | elseif strcmpi(ToDataStoreMemory,'off') && ~isempty(find_system(lib_path,'LookUnderMasks','all','FollowLinks','on','Name','AEMS_SRFLIPFLOP'))
      |     delete_block([lib_path,'/AEMS_SRFLIPFLOP']);
      |     delete_block([lib_path,'/Data Type Conversion']);
      |     delete_block([lib_path,'/Data Store Write']);
      |     delete_line(find_system(lib_path,'FollowLinks','on','FindAll','on','LookUnderMasks','on','Type','line','Connected','off'));
      | end
      | if strcmpi(ToDataStoreMemory,'on')
      |     %Get Task Rate of this block.(As per AEMS arch, all the blks shall be
      |     %kept under the runnable. The Runnable name will ncontain the sample
      |     %time suffix. From where we can get it.
      |     model_type_pos = strsplit(lib_path,'/');%to split all the layer paths in order to get the runnable path
      |     runnable_path = [bdroot '/' model_type_pos{2}];%to get the runnable or AIPCALL path
      |     trg_port_name = get_param(find_system(runnable_path,'BlockType','TriggerPort'),'Name');%to get the function call trigger name
      |     TaskRate = '';%the raster suffix is stored in the parameter
      |     
      |     if ~isempty(trg_port_name)
      |         trg_port_name_spltd = strsplit(trg_port_name{1},'_');%splitting is done in order to get the raster and its type(Sched or Event)
      |         
      |         % checking for rasters of type Sched or Event especially occuring in
      |         % runnables
      |         if ~isempty(regexp(trg_port_name_spltd{1},'^Sched|^Event','once'))
      |             TaskRate = ['_' regexprep(trg_port_name_spltd{1},'Sched|Event','','once')];
      |             
      |             %checking if the raster is dcmcb and this is applicable only for
      |             %APICALL
      |         elseif ~isempty(regexp([trg_port_name_spltd{1} '_' trg_port_name_spltd{2} '_' ],'^DataServices_DCM_|^RoutineServices_DCM_','once'))||...
      |                 ~isempty(regexp(trg_port_name_spltd{1},'^Dcm$','once'))
      |             TaskRate = '_dcmcb';
      |             
      |             %checking if this block is used under the function call trigger
      |             %starting with "Com" and then giving an error message
      |             %this is applicable only for APICALL
      |         elseif ~isempty(regexp(trg_port_name_spltd{1},'^Com$','once'))
      |             msg = sprintf(['\n','The FIM block "' lib_path '" should not be present within APICALLs having function call trigger as "Com"']);
      |             errordlg(msg);
      |             return;
      |         end
      |     end
      |     DataStoreName = [eventid,TaskRate];
      |     set_param([lib_path,'/Data Store Write'],'DataStoreName',DataStoreName);
      | end
      | Attribute_Format_String_Part5 = '\n Write Output To Data Store Memory := %<ToDataStoreMemory>';
      | 
      | Attribute_Format_String_Part4='\n Debounce Time Failed Threshold = %<DemDebounceTimeFailedThreshold>\nDebounce Time Passed Threshold = %<DemDebounceTimePassedThreshold>\nDem Debounce Time Bypass Failure = %<DemTimeBypassFailure>\nSample Time = %<sampletime>';
      | Attribute_Format_String = [Attribute_Format_String_Part1,Attribute_Format_String_Part2,Attribute_Format_String_Part3,Attribute_Format_String_Part4, Attribute_Format_String_Part5];
      | 
      | set_param(lib_path,'AttributesFormatString',Attribute_Format_String);
      settings: AttributesFormatString=%<MaskType>\n EventId : %<eventid> \n Specific case used only for Nissan cases = %<Specificchoix> \n Dem Debounce Behavior 1 = %<DemDebounceBehavior1>\n Debounce Time Failed Threshold = %<DemDebounceTimeFailedThreshold>\nDebounce Time Passed Threshold = %<DemDebounceTimePassedThreshold>\nDem Debounce Time Bypass Failure = %<DemTimeBypassFailure>\nSample Time = %<sampletime>\n Write Output To Data Store Memory := %<ToDataStoreMemory>
      mask Help:
      | eval('path_lib=fileparts(which(''AEMS_Standard_Library''));');
      | doc_path = [path_lib '\help\AEMS_DEM_TIME_BASED_DEBOUNCE.pdf'];
      | eval('open(doc_path)');
      mask Callback eventid:
      | lib_path=gcb;
      | EventID=get_param(lib_path,'eventid');
      | Splitname=regexp(EventID,'_','all');
      | EventID_Name=extractAfter(EventID,EventID(1:Splitname(2)));
      | Fail_Thrs=strcat('Cxx_dem_fail_thd_',EventID_Name);
      | set_param(lib_path,'DemDebounceTimeFailedThreshold',Fail_Thrs);
      | Pass_Thrs=strcat('Cxx_dem_pass_thd_',EventID_Name);
      | set_param(lib_path,'DemDebounceTimePassedThreshold',Pass_Thrs);
      | BypassFailure=strcat('Cbx_dem_byp_fail_',EventID_Name);
      | set_param(lib_path,'DemTimeBypassFailure',BypassFailure);
      | 
      | ToDataStoreMemory = get_param(lib_path,'ToDataStoreMemory');
      | 
      | if strcmpi(ToDataStoreMemory,'on')
      | model_type_pos = strsplit(lib_path,'/');%to split all the layer paths in order to get the runnable path
      | runnable_path = [bdroot '/' model_type_pos{2}];%to get the runnable or AIPCALL path
      | trg_port_name = get_param(find_system(runnable_path,'BlockType','TriggerPort'),'Name');%to get the function call trigger name
      | TaskRate = '';%the raster suffix is stored in the parameter
      | 
      | if ~isempty(trg_port_name)
      |     trg_port_name_spltd = strsplit(trg_port_name{1},'_');%splitting is done in order to get the raster and its type(Sched or Event)
      | 
      |     % checking for rasters of type Sched or Event especially occuring in
      |     % runnables
      |     if ~isempty(regexp(trg_port_name_spltd{1},'^Sched\d+(ms|s)$|^Event+(sync|knock|comc|coml|dcmcb)$','once'))
      |         TaskRate = ['_' regexp(trg_port_name_spltd{1},'\d+(ms|s)$|sync$|knock$|comc$|coml$|dcmcb$','match','once')];
      | 
      |     %checking if the raster is dcmcb and this is applicable only for
      |     %APICALL
      |     elseif ~isempty(regexp([trg_port_name_spltd{1} '_' trg_port_name_spltd{2} '_' ],'^DataServices_DCM_|^RoutineServices_DCM_','once'))||...
      |             ~isempty(regexp(trg_port_name_spltd{1},'^Dcm$','once'))
      |         TaskRate = '_dcmcb';
      | 
      |     %checking if this block is used under the function call trigger
      |     %starting with "Com" and then giving an error message
      |     %this is applicable only for APICALL
      |     elseif ~isempty(regexp(trg_port_name_spltd{1},'^Com$','once'))
      |         msg = sprintf(['\n','The DEM blocks "' Thisblk '" should not be present within APICALLs having function call trigger as "Com"']);
      |         errordlg(msg);
      |         return;
      |     end
      | end
      | DataStoreName = [EventID TaskRate];%the variable name that should be given to DataStoreRead block
      | set_param([lib_path,'/Data Store Write'],'DataStoreName',DataStoreName);
      | else
      |     %do nothing
      | end
      mask Callback Specificchoix:
      | Outputs_From_get_param = get_param(gcb,'Dim_num');
      | Specificchoice_get_param = get_param(gcb,'Specificchoix');
      | maskobj = Simulink.Mask.get(gcbh);
      | maskobj_param = maskobj.Parameters;
      |     if strcmpi(Specificchoice_get_param,'on')
      |        Non=4;
      |         maskobj_param(3).Visible = 'on';
